simulink model "gm_minutiaeextraction_21821"  (R2018b)
settings: Solver=FixedStepDiscrete  StartTime=0.0  StopTime=10  RelTol=1e-3
undefined symbols (not defined in the file or in its folder): gray
libraries: hdlsllib x4, visionsources x1, dspmtrx3 x1
(part 5 of 7)

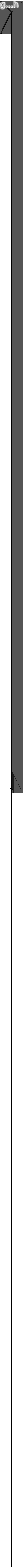
== system gm_minutiaeextraction_21821/MinutiaeFeature/MinutaeExtractTh ==
  In1 : Inport  OutDataTypeStr=boolean  PortDimensions=[128,64]  SampleTime=0.1
  MATLAB Function1 : Subsystem
  Serializer1D : hdlsllib/HDL Operations/Serializer1D  Ratio=8192  IdleCycles=0  validIn=off  startOut=off  validOut=off  inputDataDimensions=8192  inputSampleTime=0.1  inputSignalType=real
      settings: SourceProductName=HDL Coder  SourceProductBaseCode=HD
  concatenate : Concatenate  NumInputs=8192  ConcatenateDimension=2
  t : Subsystem
  t{1..64} (64 alike) : Demux  Outputs=128
  Out1 : Outport
  wires:
  In1/1 -> MATLAB Function1/1(X)
  MATLAB Function1/1(Y) -> t/1(in0)
  concatenate/1 -> Serializer1D/1
  Serializer1D/1 -> Out1/1
  t/1(out0) -> t1/1
  t/2(out1) -> t2/1
  t/3(out2) -> t3/1
  t/4(out3) -> t4/1
  t/5(out4) -> t5/1
  t/6(out5) -> t6/1
  t/7(out6) -> t7/1
  t/8(out7) -> t8/1
  t/9(out8) -> t9/1
  t/10(out9) -> t10/1
  t/11(out10) -> t11/1
  t/12(out11) -> t12/1
  t/13(out12) -> t13/1
  t/14(out13) -> t14/1
  t/15(out14) -> t15/1
  t/16(out15) -> t16/1
  t/17(out16) -> t17/1
  t/18(out17) -> t18/1
  t/19(out18) -> t19/1
  t/20(out19) -> t20/1
  t/21(out20) -> t21/1
  t/22(out21) -> t22/1
  t/23(out22) -> t23/1
  t/24(out23) -> t24/1
  t/25(out24) -> t25/1
  t/26(out25) -> t26/1
  t/27(out26) -> t27/1
  t/28(out27) -> t28/1
  t/29(out28) -> t29/1
  t/30(out29) -> t30/1
  t/31(out30) -> t31/1
  t/32(out31) -> t32/1
  t/33(out32) -> t33/1
  t/34(out33) -> t34/1
  t/35(out34) -> t35/1
  t/36(out35) -> t36/1
  t/37(out36) -> t37/1
  t/38(out37) -> t38/1
  t/39(out38) -> t39/1
  t/40(out39) -> t40/1
  t/41(out40) -> t41/1
  t/42(out41) -> t42/1
  t/43(out42) -> t43/1
  t/44(out43) -> t44/1
  t/45(out44) -> t45/1
  t/46(out45) -> t46/1
  t/47(out46) -> t47/1
  t/48(out47) -> t48/1
  t/49(out48) -> t49/1
  t/50(out49) -> t50/1
  t/51(out50) -> t51/1
  t/52(out51) -> t52/1
  t/53(out52) -> t53/1
  t/54(out53) -> t54/1
  t/55(out54) -> t55/1
  t/56(out55) -> t56/1
  t/57(out56) -> t57/1
  t/58(out57) -> t58/1
  t/59(out58) -> t59/1
  t/60(out59) -> t60/1
  t/61(out60) -> t61/1
  t/62(out61) -> t62/1
  t/63(out62) -> t63/1
  t/64(out63) -> t64/1
  t1/1 -> concatenate/1
  t1/2 -> concatenate/2
  t1/3 -> concatenate/3
  t1/4 -> concatenate/4
  t1/5 -> concatenate/5
  t1/6 -> concatenate/6
  t1/7 -> concatenate/7
  t1/8 -> concatenate/8
  t1/9 -> concatenate/9
  t1/10 -> concatenate/10
  t1/11 -> concatenate/11
  t1/12 -> concatenate/12
  t1/13 -> concatenate/13
  t1/14 -> concatenate/14
  t1/15 -> concatenate/15
  t1/16 -> concatenate/16
  t1/17 -> concatenate/17
  t1/18 -> concatenate/18
  t1/19 -> concatenate/19
  t1/20 -> concatenate/20
  t1/21 -> concatenate/21
  t1/22 -> concatenate/22
  t1/23 -> concatenate/23
  t1/24 -> concatenate/24
  t1/25 -> concatenate/25
  t1/26 -> concatenate/26
  t1/27 -> concatenate/27
  t1/28 -> concatenate/28
  t1/29 -> concatenate/29
  t1/30 -> concatenate/30
  t1/31 -> concatenate/31
  t1/32 -> concatenate/32
  t1/33 -> concatenate/33
  t1/34 -> concatenate/34
  t1/35 -> concatenate/35
  t1/36 -> concatenate/36
  t1/37 -> concatenate/37
  t1/38 -> concatenate/38
  t1/39 -> concatenate/39
  t1/40 -> concatenate/40
  t1/41 -> concatenate/41
  t1/42 -> concatenate/42
  t1/43 -> concatenate/43
  t1/44 -> concatenate/44
  t1/45 -> concatenate/45
  t1/46 -> concatenate/46
  t1/47 -> concatenate/47
  t1/48 -> concatenate/48
  t1/49 -> concatenate/49
  t1/50 -> concatenate/50
  t1/51 -> concatenate/51
  t1/52 -> concatenate/52
  t1/53 -> concatenate/53
  t1/54 -> concatenate/54
  t1/55 -> concatenate/55
  t1/56 -> concatenate/56
  t1/57 -> concatenate/57
  t1/58 -> concatenate/58
  t1/59 -> concatenate/59
  t1/60 -> concatenate/60
  t1/61 -> concatenate/61
  t1/62 -> concatenate/62
  t1/63 -> concatenate/63
  t1/64 -> concatenate/64
  t1/65 -> concatenate/65
  t1/66 -> concatenate/66
  t1/67 -> concatenate/67
  t1/68 -> concatenate/68
  t1/69 -> concatenate/69
  t1/70 -> concatenate/70
  t1/71 -> concatenate/71
  t1/72 -> concatenate/72
  t1/73 -> concatenate/73
  t1/74 -> concatenate/74
  t1/75 -> concatenate/75
  t1/76 -> concatenate/76
  t1/77 -> concatenate/77
  t1/78 -> concatenate/78
  t1/79 -> concatenate/79
  t1/80 -> concatenate/80
  t1/81 -> concatenate/81
  t1/82 -> concatenate/82
  t1/83 -> concatenate/83
  t1/84 -> concatenate/84
  t1/85 -> concatenate/85
  t1/86 -> concatenate/86
  t1/87 -> concatenate/87
  t1/88 -> concatenate/88
  t1/89 -> concatenate/89
  t1/90 -> concatenate/90
  t1/91 -> concatenate/91
  t1/92 -> concatenate/92
  t1/93 -> concatenate/93
  t1/94 -> concatenate/94
  t1/95 -> concatenate/95
  t1/96 -> concatenate/96
  t1/97 -> concatenate/97
  t1/98 -> concatenate/98
  t1/99 -> concatenate/99
  t1/100 -> concatenate/100
  t1/101 -> concatenate/101
  t1/102 -> concatenate/102
  t1/103 -> concatenate/103
  t1/104 -> concatenate/104
  t1/105 -> concatenate/105
  t1/106 -> concatenate/106
  t1/107 -> concatenate/107
  t1/108 -> concatenate/108
  t1/109 -> concatenate/109
  t1/110 -> concatenate/110
  t1/111 -> concatenate/111
  t1/112 -> concatenate/112
  t1/113 -> concatenate/113
  t1/114 -> concatenate/114
  t1/115 -> concatenate/115
  t1/116 -> concatenate/116
  t1/117 -> concatenate/117
  t1/118 -> concatenate/118
  t1/119 -> concatenate/119
  t1/120 -> concatenate/120
  t1/121 -> concatenate/121
  t1/122 -> concatenate/122
  t1/123 -> concatenate/123
  t1/124 -> concatenate/124
  t1/125 -> concatenate/125
  t1/126 -> concatenate/126
  t1/127 -> concatenate/127
  t1/128 -> concatenate/128
  t2/1 -> concatenate/129
  t2/2 -> concatenate/130
  t2/3 -> concatenate/131
  t2/4 -> concatenate/132
  t2/5 -> concatenate/133
  t2/6 -> concatenate/134
  t2/7 -> concatenate/135
  t2/8 -> concatenate/136
  t2/9 -> concatenate/137
  t2/10 -> concatenate/138
  t2/11 -> concatenate/139
  t2/12 -> concatenate/140
  t2/13 -> concatenate/141
  t2/14 -> concatenate/142
  t2/15 -> concatenate/143
  t2/16 -> concatenate/144
  t2/17 -> concatenate/145
  t2/18 -> concatenate/146
  t2/19 -> concatenate/147
  t2/20 -> concatenate/148
  t2/21 -> concatenate/149
  t2/22 -> concatenate/150
  t2/23 -> concatenate/151
  t2/24 -> concatenate/152
  t2/25 -> concatenate/153
  t2/26 -> concatenate/154
  t2/27 -> concatenate/155
  t2/28 -> concatenate/156
  t2/29 -> concatenate/157
  t2/30 -> concatenate/158
  t2/31 -> concatenate/159
  t2/32 -> concatenate/160
  t2/33 -> concatenate/161
  t2/34 -> concatenate/162
  t2/35 -> concatenate/163
  t2/36 -> concatenate/164
  t2/37 -> concatenate/165
  t2/38 -> concatenate/166
  t2/39 -> concatenate/167
  t2/40 -> concatenate/168
  t2/41 -> concatenate/169
  t2/42 -> concatenate/170
  t2/43 -> concatenate/171
  t2/44 -> concatenate/172
  t2/45 -> concatenate/173
  t2/46 -> concatenate/174
  t2/47 -> concatenate/175
  t2/48 -> concatenate/176
  t2/49 -> concatenate/177
  t2/50 -> concatenate/178
  t2/51 -> concatenate/179
  t2/52 -> concatenate/180
  t2/53 -> concatenate/181
  t2/54 -> concatenate/182
  t2/55 -> concatenate/183
  t2/56 -> concatenate/184
  t2/57 -> concatenate/185
  t2/58 -> concatenate/186
  t2/59 -> concatenate/187
  t2/60 -> concatenate/188
  t2/61 -> concatenate/189
  t2/62 -> concatenate/190
  t2/63 -> concatenate/191
  t2/64 -> concatenate/192
  t2/65 -> concatenate/193
  t2/66 -> concatenate/194
  t2/67 -> concatenate/195
  t2/68 -> concatenate/196
  t2/69 -> concatenate/197
  t2/70 -> concatenate/198
  t2/71 -> concatenate/199
  t2/72 -> concatenate/200
  t2/73 -> concatenate/201
  t2/74 -> concatenate/202
  t2/75 -> concatenate/203
  t2/76 -> concatenate/204
  t2/77 -> concatenate/205
  t2/78 -> concatenate/206
  t2/79 -> concatenate/207
  t2/80 -> concatenate/208
  t2/81 -> concatenate/209
  t2/82 -> concatenate/210
  t2/83 -> concatenate/211
  t2/84 -> concatenate/212
  t2/85 -> concatenate/213
  t2/86 -> concatenate/214
  t2/87 -> concatenate/215
  t2/88 -> concatenate/216
  t2/89 -> concatenate/217
  t2/90 -> concatenate/218
  t2/91 -> concatenate/219
  t2/92 -> concatenate/220
  t2/93 -> concatenate/221
  t2/94 -> concatenate/222
  t2/95 -> concatenate/223
  t2/96 -> concatenate/224
  t2/97 -> concatenate/225
  t2/98 -> concatenate/226
  t2/99 -> concatenate/227
  t2/100 -> concatenate/228
  t2/101 -> concatenate/229
  t2/102 -> concatenate/230
  t2/103 -> concatenate/231
  t2/104 -> concatenate/232
  t2/105 -> concatenate/233
  t2/106 -> concatenate/234
  t2/107 -> concatenate/235
  t2/108 -> concatenate/236
  t2/109 -> concatenate/237
  t2/110 -> concatenate/238
  t2/111 -> concatenate/239
  t2/112 -> concatenate/240
  t2/113 -> concatenate/241
  t2/114 -> concatenate/242
  t2/115 -> concatenate/243
  t2/116 -> concatenate/244
  t2/117 -> concatenate/245
  t2/118 -> concatenate/246
  t2/119 -> concatenate/247
  t2/120 -> concatenate/248
  t2/121 -> concatenate/249
  t2/122 -> concatenate/250
  t2/123 -> concatenate/251
  t2/124 -> concatenate/252
  t2/125 -> concatenate/253
  t2/126 -> concatenate/254
  t2/127 -> concatenate/255
  t2/128 -> concatenate/256
  t3/1 -> concatenate/257
  t3/2 -> concatenate/258
  t3/3 -> concatenate/259
  t3/4 -> concatenate/260
  t3/5 -> concatenate/261
  t3/6 -> concatenate/262
  t3/7 -> concatenate/263
  t3/8 -> concatenate/264
  t3/9 -> concatenate/265
  t3/10 -> concatenate/266
  t3/11 -> concatenate/267
  t3/12 -> concatenate/268
  t3/13 -> concatenate/269
  t3/14 -> concatenate/270
  t3/15 -> concatenate/271
  t3/16 -> concatenate/272
  t3/17 -> concatenate/273
  t3/18 -> concatenate/274
  t3/19 -> concatenate/275
  t3/20 -> concatenate/276
  t3/21 -> concatenate/277
  t3/22 -> concatenate/278
  t3/23 -> concatenate/279
  t3/24 -> concatenate/280
  t3/25 -> concatenate/281
  t3/26 -> concatenate/282
  t3/27 -> concatenate/283
  t3/28 -> concatenate/284
  t3/29 -> concatenate/285
  t3/30 -> concatenate/286
  t3/31 -> concatenate/287
  t3/32 -> concatenate/288
  t3/33 -> concatenate/289
  t3/34 -> concatenate/290
  t3/35 -> concatenate/291
  t3/36 -> concatenate/292
  t3/37 -> concatenate/293
  t3/38 -> concatenate/294
  t3/39 -> concatenate/295
  t3/40 -> concatenate/296
  t3/41 -> concatenate/297
  t3/42 -> concatenate/298
  t3/43 -> concatenate/299
  t3/44 -> concatenate/300
  t3/45 -> concatenate/301
  t3/46 -> concatenate/302
  t3/47 -> concatenate/303
  t3/48 -> concatenate/304
  t3/49 -> concatenate/305
  t3/50 -> concatenate/306
  t3/51 -> concatenate/307
  t3/52 -> concatenate/308
  t3/53 -> concatenate/309
  t3/54 -> concatenate/310
  t3/55 -> concatenate/311
  t3/56 -> concatenate/312
  t3/57 -> concatenate/313
  t3/58 -> concatenate/314
  t3/59 -> concatenate/315
  t3/60 -> concatenate/316
  t3/61 -> concatenate/317
  t3/62 -> concatenate/318
  t3/63 -> concatenate/319
  t3/64 -> concatenate/320
  t3/65 -> concatenate/321
  t3/66 -> concatenate/322
  t3/67 -> concatenate/323
  t3/68 -> concatenate/324
  t3/69 -> concatenate/325
  t3/70 -> concatenate/326
  t3/71 -> concatenate/327
  t3/72 -> concatenate/328
  t3/73 -> concatenate/329
  t3/74 -> concatenate/330
  t3/75 -> concatenate/331
  t3/76 -> concatenate/332
  t3/77 -> concatenate/333
  t3/78 -> concatenate/334
  t3/79 -> concatenate/335
  t3/80 -> concatenate/336
  t3/81 -> concatenate/337
  t3/82 -> concatenate/338
  t3/83 -> concatenate/339
  t3/84 -> concatenate/340
  t3/85 -> concatenate/341
  t3/86 -> concatenate/342
  t3/87 -> concatenate/343
  t3/88 -> concatenate/344
  t3/89 -> concatenate/345
  t3/90 -> concatenate/346
  t3/91 -> concatenate/347
  t3/92 -> concatenate/348
  t3/93 -> concatenate/349
  t3/94 -> concatenate/350
  t3/95 -> concatenate/351
  t3/96 -> concatenate/352
  t3/97 -> concatenate/353
  t3/98 -> concatenate/354
  t3/99 -> concatenate/355
  t3/100 -> concatenate/356
  t3/101 -> concatenate/357
  t3/102 -> concatenate/358
  t3/103 -> concatenate/359
  t3/104 -> concatenate/360
  t3/105 -> concatenate/361
  t3/106 -> concatenate/362
  t3/107 -> concatenate/363
  t3/108 -> concatenate/364
  t3/109 -> concatenate/365
  t3/110 -> concatenate/366
  t3/111 -> concatenate/367
  t3/112 -> concatenate/368
  t3/113 -> concatenate/369
  t3/114 -> concatenate/370
  t3/115 -> concatenate/371
  t3/116 -> concatenate/372
  t3/117 -> concatenate/373
  t3/118 -> concatenate/374
  t3/119 -> concatenate/375
  t3/120 -> concatenate/376
  t3/121 -> concatenate/377
  t3/122 -> concatenate/378
  t3/123 -> concatenate/379
  t3/124 -> concatenate/380
  t3/125 -> concatenate/381
  t3/126 -> concatenate/382
  t3/127 -> concatenate/383
  t3/128 -> concatenate/384
  t4/1 -> concatenate/385
  t4/2 -> concatenate/386
  t4/3 -> concatenate/387
  t4/4 -> concatenate/388
  t4/5 -> concatenate/389
  t4/6 -> concatenate/390
  t4/7 -> concatenate/391
  t4/8 -> concatenate/392
  t4/9 -> concatenate/393
  t4/10 -> concatenate/394
  t4/11 -> concatenate/395
  t4/12 -> concatenate/396
  t4/13 -> concatenate/397
  t4/14 -> concatenate/398
  t4/15 -> concatenate/399
  t4/16 -> concatenate/400
  t4/17 -> concatenate/401
  t4/18 -> concatenate/402
  t4/19 -> concatenate/403
  t4/20 -> concatenate/404
  t4/21 -> concatenate/405
  t4/22 -> concatenate/406
  t4/23 -> concatenate/407
  t4/24 -> concatenate/408
  t4/25 -> concatenate/409
  t4/26 -> concatenate/410
  t4/27 -> concatenate/411
  t4/28 -> concatenate/412
  t4/29 -> concatenate/413
  t4/30 -> concatenate/414
  t4/31 -> concatenate/415
  t4/32 -> concatenate/416
  t4/33 -> concatenate/417
  t4/34 -> concatenate/418
  t4/35 -> concatenate/419
  t4/36 -> concatenate/420
  t4/37 -> concatenate/421
  t4/38 -> concatenate/422
  t4/39 -> concatenate/423
  t4/40 -> concatenate/424
  t4/41 -> concatenate/425
  t4/42 -> concatenate/426
  t4/43 -> concatenate/427
  t4/44 -> concatenate/428
  t4/45 -> concatenate/429
  t4/46 -> concatenate/430
  t4/47 -> concatenate/431
  t4/48 -> concatenate/432
  t4/49 -> concatenate/433
  t4/50 -> concatenate/434
  t4/51 -> concatenate/435
  t4/52 -> concatenate/436
  t4/53 -> concatenate/437
  t4/54 -> concatenate/438
  t4/55 -> concatenate/439
  t4/56 -> concatenate/440
  t4/57 -> concatenate/441
  t4/58 -> concatenate/442
  t4/59 -> concatenate/443
  t4/60 -> concatenate/444
  t4/61 -> concatenate/445
  t4/62 -> concatenate/446
  t4/63 -> concatenate/447
  t4/64 -> concatenate/448
  t4/65 -> concatenate/449
  t4/66 -> concatenate/450
  t4/67 -> concatenate/451
  t4/68 -> concatenate/452
  t4/69 -> concatenate/453
  t4/70 -> concatenate/454
  t4/71 -> concatenate/455
  t4/72 -> concatenate/456
  t4/73 -> concatenate/457
  t4/74 -> concatenate/458
  t4/75 -> concatenate/459
  t4/76 -> concatenate/460
  t4/77 -> concatenate/461
  t4/78 -> concatenate/462
  t4/79 -> concatenate/463
  t4/80 -> concatenate/464
  t4/81 -> concatenate/465
  t4/82 -> concatenate/466
  t4/83 -> concatenate/467
  t4/84 -> concatenate/468
  t4/85 -> concatenate/469
  t4/86 -> concatenate/470
  t4/87 -> concatenate/471
  t4/88 -> concatenate/472
  t4/89 -> concatenate/473
  t4/90 -> concatenate/474
  t4/91 -> concatenate/475
  t4/92 -> concatenate/476
  t4/93 -> concatenate/477
  t4/94 -> concatenate/478
  t4/95 -> concatenate/479
  t4/96 -> concatenate/480
  t4/97 -> concatenate/481
  t4/98 -> concatenate/482
  t4/99 -> concatenate/483
  t4/100 -> concatenate/484
  t4/101 -> concatenate/485
  t4/102 -> concatenate/486
  t4/103 -> concatenate/487
  t4/104 -> concatenate/488
  t4/105 -> concatenate/489
  t4/106 -> concatenate/490
  t4/107 -> concatenate/491
  t4/108 -> concatenate/492
  t4/109 -> concatenate/493
  t4/110 -> concatenate/494
  t4/111 -> concatenate/495
  t4/112 -> concatenate/496
  t4/113 -> concatenate/497
  t4/114 -> concatenate/498
  t4/115 -> concatenate/499
  t4/116 -> concatenate/500
  t4/117 -> concatenate/501
  t4/118 -> concatenate/502
  t4/119 -> concatenate/503
  t4/120 -> concatenate/504
  t4/121 -> concatenate/505
  t4/122 -> concatenate/506
  t4/123 -> concatenate/507
  t4/124 -> concatenate/508
  t4/125 -> concatenate/509
  t4/126 -> concatenate/510
  t4/127 -> concatenate/511
  t4/128 -> concatenate/512
  t5/1 -> concatenate/513
  t5/2 -> concatenate/514
  t5/3 -> concatenate/515
  t5/4 -> concatenate/516
  t5/5 -> concatenate/517
  t5/6 -> concatenate/518
  t5/7 -> concatenate/519
  t5/8 -> concatenate/520
  t5/9 -> concatenate/521
  t5/10 -> concatenate/522
  t5/11 -> concatenate/523
  t5/12 -> concatenate/524
  t5/13 -> concatenate/525
  t5/14 -> concatenate/526
  t5/15 -> concatenate/527
  t5/16 -> concatenate/528
  t5/17 -> concatenate/529
  t5/18 -> concatenate/530
  t5/19 -> concatenate/531
  t5/20 -> concatenate/532
  t5/21 -> concatenate/533
  t5/22 -> concatenate/534
  t5/23 -> concatenate/535
  t5/24 -> concatenate/536
  t5/25 -> concatenate/537
  t5/26 -> concatenate/538
  t5/27 -> concatenate/539
  t5/28 -> concatenate/540
  t5/29 -> concatenate/541
  t5/30 -> concatenate/542
  t5/31 -> concatenate/543
  t5/32 -> concatenate/544
  t5/33 -> concatenate/545
  t5/34 -> concatenate/546
  t5/35 -> concatenate/547
  t5/36 -> concatenate/548
  t5/37 -> concatenate/549
  t5/38 -> concatenate/550
  t5/39 -> concatenate/551
  t5/40 -> concatenate/552
  t5/41 -> concatenate/553
  t5/42 -> concatenate/554
  t5/43 -> concatenate/555
  t5/44 -> concatenate/556
  t5/45 -> concatenate/557
  t5/46 -> concatenate/558
  t5/47 -> concatenate/559
  t5/48 -> concatenate/560
  t5/49 -> concatenate/561
  t5/50 -> concatenate/562
  t5/51 -> concatenate/563
  t5/52 -> concatenate/564
  t5/53 -> concatenate/565
  t5/54 -> concatenate/566
  t5/55 -> concatenate/567
  t5/56 -> concatenate/568
  t5/57 -> concatenate/569
  t5/58 -> concatenate/570
  t5/59 -> concatenate/571
  t5/60 -> concatenate/572
  t5/61 -> concatenate/573
  t5/62 -> concatenate/574
  t5/63 -> concatenate/575
  t5/64 -> concatenate/576
  t5/65 -> concatenate/577
  t5/66 -> concatenate/578
  t5/67 -> concatenate/579
  t5/68 -> concatenate/580
  t5/69 -> concatenate/581
  t5/70 -> concatenate/582
  t5/71 -> concatenate/583
  t5/72 -> concatenate/584
  t5/73 -> concatenate/585
  t5/74 -> concatenate/586
  t5/75 -> concatenate/587
  t5/76 -> concatenate/588
  t5/77 -> concatenate/589
  t5/78 -> concatenate/590
  t5/79 -> concatenate/591
  t5/80 -> concatenate/592
  t5/81 -> concatenate/593
  t5/82 -> concatenate/594
  t5/83 -> concatenate/595
  t5/84 -> concatenate/596
  t5/85 -> concatenate/597
  t5/86 -> concatenate/598
  t5/87 -> concatenate/599
  t5/88 -> concatenate/600
  t5/89 -> concatenate/601
  t5/90 -> concatenate/602
  t5/91 -> concatenate/603
  t5/92 -> concatenate/604
  t5/93 -> concatenate/605
  t5/94 -> concatenate/606
  t5/95 -> concatenate/607
  t5/96 -> concatenate/608
  t5/97 -> concatenate/609
  t5/98 -> concatenate/610
  t5/99 -> concatenate/611
  t5/100 -> concatenate/612
  t5/101 -> concatenate/613
  t5/102 -> concatenate/614
  t5/103 -> concatenate/615
  t5/104 -> concatenate/616
  t5/105 -> concatenate/617
  t5/106 -> concatenate/618
  t5/107 -> concatenate/619
  t5/108 -> concatenate/620
  t5/109 -> concatenate/621
  t5/110 -> concatenate/622
  t5/111 -> concatenate/623
  t5/112 -> concatenate/624
  t5/113 -> concatenate/625
  t5/114 -> concatenate/626
  t5/115 -> concatenate/627
  t5/116 -> concatenate/628
  t5/117 -> concatenate/629
  t5/118 -> concatenate/630
  t5/119 -> concatenate/631
  t5/120 -> concatenate/632
  t5/121 -> concatenate/633
  t5/122 -> concatenate/634
  t5/123 -> concatenate/635
  t5/124 -> concatenate/636
  t5/125 -> concatenate/637
  t5/126 -> concatenate/638
  t5/127 -> concatenate/639
  t5/128 -> concatenate/640
  t6/1 -> concatenate/641
  t6/2 -> concatenate/642
  t6/3 -> concatenate/643
  t6/4 -> concatenate/644
  t6/5 -> concatenate/645
  t6/6 -> concatenate/646
  t6/7 -> concatenate/647
  t6/8 -> concatenate/648
  t6/9 -> concatenate/649
  t6/10 -> concatenate/650
  t6/11 -> concatenate/651
  t6/12 -> concatenate/652
  t6/13 -> concatenate/653
  t6/14 -> concatenate/654
  t6/15 -> concatenate/655
  t6/16 -> concatenate/656
  t6/17 -> concatenate/657
  t6/18 -> concatenate/658
  t6/19 -> concatenate/659
  t6/20 -> concatenate/660
  t6/21 -> concatenate/661
  t6/22 -> concatenate/662
  t6/23 -> concatenate/663
  t6/24 -> concatenate/664
  t6/25 -> concatenate/665
  t6/26 -> concatenate/666
  t6/27 -> concatenate/667
  t6/28 -> concatenate/668
  t6/29 -> concatenate/669
  t6/30 -> concatenate/670
  t6/31 -> concatenate/671
  t6/32 -> concatenate/672
  t6/33 -> concatenate/673
  t6/34 -> concatenate/674
  t6/35 -> concatenate/675
  t6/36 -> concatenate/676
  t6/37 -> concatenate/677
  t6/38 -> concatenate/678
  t6/39 -> concatenate/679
  t6/40 -> concatenate/680
  t6/41 -> concatenate/681
  t6/42 -> concatenate/682
  t6/43 -> concatenate/683
  t6/44 -> concatenate/684
  t6/45 -> concatenate/685
  t6/46 -> concatenate/686
  t6/47 -> concatenate/687
  t6/48 -> concatenate/688
  t6/49 -> concatenate/689
  t6/50 -> concatenate/690
  t6/51 -> concatenate/691
  t6/52 -> concatenate/692
  t6/53 -> concatenate/693
  t6/54 -> concatenate/694
  t6/55 -> concatenate/695
  t6/56 -> concatenate/696
  t6/57 -> concatenate/697
  t6/58 -> concatenate/698
  t6/59 -> concatenate/699
  t6/60 -> concatenate/700
  t6/61 -> concatenate/701
  t6/62 -> concatenate/702
  t6/63 -> concatenate/703
  t6/64 -> concatenate/704
  t6/65 -> concatenate/705
  t6/66 -> concatenate/706
  t6/67 -> concatenate/707
  t6/68 -> concatenate/708
  t6/69 -> concatenate/709
  t6/70 -> concatenate/710
  t6/71 -> concatenate/711
  t6/72 -> concatenate/712
  t6/73 -> concatenate/713
  t6/74 -> concatenate/714
  t6/75 -> concatenate/715
  t6/76 -> concatenate/716
  t6/77 -> concatenate/717
  t6/78 -> concatenate/718
  t6/79 -> concatenate/719
  t6/80 -> concatenate/720
  t6/81 -> concatenate/721
  t6/82 -> concatenate/722
  t6/83 -> concatenate/723
  t6/84 -> concatenate/724
  t6/85 -> concatenate/725
  t6/86 -> concatenate/726
  t6/87 -> concatenate/727
  t6/88 -> concatenate/728
  t6/89 -> concatenate/729
  t6/90 -> concatenate/730
  t6/91 -> concatenate/731
  t6/92 -> concatenate/732
  t6/93 -> concatenate/733
  t6/94 -> concatenate/734
  t6/95 -> concatenate/735
  t6/96 -> concatenate/736
  t6/97 -> concatenate/737
  t6/98 -> concatenate/738
  t6/99 -> concatenate/739
  t6/100 -> concatenate/740
  t6/101 -> concatenate/741
  t6/102 -> concatenate/742
  t6/103 -> concatenate/743
  t6/104 -> concatenate/744
  t6/105 -> concatenate/745
  t6/106 -> concatenate/746
  t6/107 -> concatenate/747
  t6/108 -> concatenate/748
  t6/109 -> concatenate/749
  t6/110 -> concatenate/750
  t6/111 -> concatenate/751
  t6/112 -> concatenate/752
  t6/113 -> concatenate/753
  t6/114 -> concatenate/754
  t6/115 -> concatenate/755
  t6/116 -> concatenate/756
  t6/117 -> concatenate/757
  t6/118 -> concatenate/758
  t6/119 -> concatenate/759
  t6/120 -> concatenate/760
  t6/121 -> concatenate/761
  t6/122 -> concatenate/762
  t6/123 -> concatenate/763
  t6/124 -> concatenate/764
  t6/125 -> concatenate/765
  t6/126 -> concatenate/766
  t6/127 -> concatenate/767
  t6/128 -> concatenate/768
  t7/1 -> concatenate/769
  t7/2 -> concatenate/770
  t7/3 -> concatenate/771
  t7/4 -> concatenate/772
  t7/5 -> concatenate/773
  t7/6 -> concatenate/774
  t7/7 -> concatenate/775
  t7/8 -> concatenate/776
  t7/9 -> concatenate/777
  t7/10 -> concatenate/778
  t7/11 -> concatenate/779
  t7/12 -> concatenate/780
  t7/13 -> concatenate/781
  t7/14 -> concatenate/782
  t7/15 -> concatenate/783
  t7/16 -> concatenate/784
  t7/17 -> concatenate/785
  t7/18 -> concatenate/786
  t7/19 -> concatenate/787
  t7/20 -> concatenate/788
  t7/21 -> concatenate/789
  t7/22 -> concatenate/790
  t7/23 -> concatenate/791
  t7/24 -> concatenate/792
  t7/25 -> concatenate/793
  t7/26 -> concatenate/794
  t7/27 -> concatenate/795
  t7/28 -> concatenate/796
  t7/29 -> concatenate/797
  t7/30 -> concatenate/798
  t7/31 -> concatenate/799
  t7/32 -> concatenate/800
  t7/33 -> concatenate/801
  t7/34 -> concatenate/802
  t7/35 -> concatenate/803
  t7/36 -> concatenate/804
  t7/37 -> concatenate/805
  t7/38 -> concatenate/806
  t7/39 -> concatenate/807
  t7/40 -> concatenate/808
  t7/41 -> concatenate/809
  t7/42 -> concatenate/810
  t7/43 -> concatenate/811
  t7/44 -> concatenate/812
  t7/45 -> concatenate/813
  t7/46 -> concatenate/814
  t7/47 -> concatenate/815
  t7/48 -> concatenate/816
  t7/49 -> concatenate/817
  t7/50 -> concatenate/818
  t7/51 -> concatenate/819
  t7/52 -> concatenate/820
  t7/53 -> concatenate/821
  t7/54 -> concatenate/822
  t7/55 -> concatenate/823
  t7/56 -> concatenate/824
  t7/57 -> concatenate/825
  t7/58 -> concatenate/826
  t7/59 -> concatenate/827
  t7/60 -> concatenate/828
  t7/61 -> concatenate/829
  t7/62 -> concatenate/830
  t7/63 -> concatenate/831
  t7/64 -> concatenate/832
  t7/65 -> concatenate/833
  t7/66 -> concatenate/834
  t7/67 -> concatenate/835
  t7/68 -> concatenate/836
  t7/69 -> concatenate/837
  t7/70 -> concatenate/838
  t7/71 -> concatenate/839
  t7/72 -> concatenate/840
  t7/73 -> concatenate/841
  t7/74 -> concatenate/842
  t7/75 -> concatenate/843
  t7/76 -> concatenate/844
  t7/77 -> concatenate/845
  t7/78 -> concatenate/846
  t7/79 -> concatenate/847
  t7/80 -> concatenate/848
  t7/81 -> concatenate/849
  t7/82 -> concatenate/850
  t7/83 -> concatenate/851
  t7/84 -> concatenate/852
  t7/85 -> concatenate/853
  t7/86 -> concatenate/854
  t7/87 -> concatenate/855
  t7/88 -> concatenate/856
  t7/89 -> concatenate/857
  t7/90 -> concatenate/858
  t7/91 -> concatenate/859
  t7/92 -> concatenate/860
  t7/93 -> concatenate/861
  t7/94 -> concatenate/862
  t7/95 -> concatenate/863
  t7/96 -> concatenate/864
  t7/97 -> concatenate/865
  t7/98 -> concatenate/866
  t7/99 -> concatenate/867
  t7/100 -> concatenate/868
  t7/101 -> concatenate/869
  t7/102 -> concatenate/870
  t7/103 -> concatenate/871
  t7/104 -> concatenate/872
  t7/105 -> concatenate/873
  t7/106 -> concatenate/874
  t7/107 -> concatenate/875
  t7/108 -> concatenate/876
  t7/109 -> concatenate/877
  t7/110 -> concatenate/878
  t7/111 -> concatenate/879
  t7/112 -> concatenate/880
  t7/113 -> concatenate/881
  t7/114 -> concatenate/882
  t7/115 -> concatenate/883
  t7/116 -> concatenate/884
  t7/117 -> concatenate/885
  t7/118 -> concatenate/886
  t7/119 -> concatenate/887
  t7/120 -> concatenate/888
  t7/121 -> concatenate/889
  t7/122 -> concatenate/890
  t7/123 -> concatenate/891
  t7/124 -> concatenate/892
  t7/125 -> concatenate/893
  t7/126 -> concatenate/894
  t7/127 -> concatenate/895
  t7/128 -> concatenate/896
  t8/1 -> concatenate/897
  t8/2 -> concatenate/898
  t8/3 -> concatenate/899
  t8/4 -> concatenate/900
  t8/5 -> concatenate/901
  t8/6 -> concatenate/902
  t8/7 -> concatenate/903
  t8/8 -> concatenate/904
  t8/9 -> concatenate/905
  t8/10 -> concatenate/906
  t8/11 -> concatenate/907
  t8/12 -> concatenate/908
  t8/13 -> concatenate/909
  t8/14 -> concatenate/910
  t8/15 -> concatenate/911
  t8/16 -> concatenate/912
  t8/17 -> concatenate/913
  t8/18 -> concatenate/914
  t8/19 -> concatenate/915
  t8/20 -> concatenate/916
  t8/21 -> concatenate/917
  t8/22 -> concatenate/918
  t8/23 -> concatenate/919
  t8/24 -> concatenate/920
  t8/25 -> concatenate/921
  t8/26 -> concatenate/922
  t8/27 -> concatenate/923
  t8/28 -> concatenate/924
  t8/29 -> concatenate/925
  t8/30 -> concatenate/926
  t8/31 -> concatenate/927
  t8/32 -> concatenate/928
  t8/33 -> concatenate/929
  t8/34 -> concatenate/930
  t8/35 -> concatenate/931
  t8/36 -> concatenate/932
  t8/37 -> concatenate/933
  t8/38 -> concatenate/934
  t8/39 -> concatenate/935
  t8/40 -> concatenate/936
  t8/41 -> concatenate/937
  t8/42 -> concatenate/938
  t8/43 -> concatenate/939
  t8/44 -> concatenate/940
  t8/45 -> concatenate/941
  t8/46 -> concatenate/942
  t8/47 -> concatenate/943
  t8/48 -> concatenate/944
  t8/49 -> concatenate/945
  t8/50 -> concatenate/946
  t8/51 -> concatenate/947
  t8/52 -> concatenate/948
  t8/53 -> concatenate/949
  t8/54 -> concatenate/950
  t8/55 -> concatenate/951
  t8/56 -> concatenate/952
  t8/57 -> concatenate/953
  t8/58 -> concatenate/954
  t8/59 -> concatenate/955
  t8/60 -> concatenate/956
  t8/61 -> concatenate/957
  t8/62 -> concatenate/958
  t8/63 -> concatenate/959
  t8/64 -> concatenate/960
  t8/65 -> concatenate/961
  t8/66 -> concatenate/962
  t8/67 -> concatenate/963
  t8/68 -> concatenate/964
  t8/69 -> concatenate/965
  t8/70 -> concatenate/966
  t8/71 -> concatenate/967
  t8/72 -> concatenate/968
  t8/73 -> concatenate/969
  t8/74 -> concatenate/970
  t8/75 -> concatenate/971
  t8/76 -> concatenate/972
  t8/77 -> concatenate/973
  t8/78 -> concatenate/974
  t8/79 -> concatenate/975
  t8/80 -> concatenate/976
  t8/81 -> concatenate/977
  t8/82 -> concatenate/978
  t8/83 -> concatenate/979
  t8/84 -> concatenate/980
  t8/85 -> concatenate/981
  t8/86 -> concatenate/982
  t8/87 -> concatenate/983
  t8/88 -> concatenate/984
  t8/89 -> concatenate/985
  t8/90 -> concatenate/986
  t8/91 -> concatenate/987
  t8/92 -> concatenate/988
  t8/93 -> concatenate/989
  t8/94 -> concatenate/990
  t8/95 -> concatenate/991
  t8/96 -> concatenate/992
  t8/97 -> concatenate/993
  t8/98 -> concatenate/994
  t8/99 -> concatenate/995
  t8/100 -> concatenate/996
  t8/101 -> concatenate/997
  t8/102 -> concatenate/998
  t8/103 -> concatenate/999
  t8/104 -> concatenate/1000
  t8/105 -> concatenate/1001
  t8/106 -> concatenate/1002
  t8/107 -> concatenate/1003
  t8/108 -> concatenate/1004
  t8/109 -> concatenate/1005
  t8/110 -> concatenate/1006
  t8/111 -> concatenate/1007
  t8/112 -> concatenate/1008
  t8/113 -> concatenate/1009
  t8/114 -> concatenate/1010
  t8/115 -> concatenate/1011
  t8/116 -> concatenate/1012
  t8/117 -> concatenate/1013
  t8/118 -> concatenate/1014
  t8/119 -> concatenate/1015
  t8/120 -> concatenate/1016
  t8/121 -> concatenate/1017
  t8/122 -> concatenate/1018
  t8/123 -> concatenate/1019
  t8/124 -> concatenate/1020
  t8/125 -> concatenate/1021
  t8/126 -> concatenate/1022
  t8/127 -> concatenate/1023
  t8/128 -> concatenate/1024
  t9/1 -> concatenate/1025
  t9/2 -> concatenate/1026
  t9/3 -> concatenate/1027
  t9/4 -> concatenate/1028
  t9/5 -> concatenate/1029
  t9/6 -> concatenate/1030
  t9/7 -> concatenate/1031
  t9/8 -> concatenate/1032
  t9/9 -> concatenate/1033
  t9/10 -> concatenate/1034
  t9/11 -> concatenate/1035
  t9/12 -> concatenate/1036
  t9/13 -> concatenate/1037
  t9/14 -> concatenate/1038
  t9/15 -> concatenate/1039
  t9/16 -> concatenate/1040
  t9/17 -> concatenate/1041
  t9/18 -> concatenate/1042
  t9/19 -> concatenate/1043
  t9/20 -> concatenate/1044
  t9/21 -> concatenate/1045
  t9/22 -> concatenate/1046
  t9/23 -> concatenate/1047
  t9/24 -> concatenate/1048
  t9/25 -> concatenate/1049
  t9/26 -> concatenate/1050
  t9/27 -> concatenate/1051
  t9/28 -> concatenate/1052
  t9/29 -> concatenate/1053
  t9/30 -> concatenate/1054
  t9/31 -> concatenate/1055
  t9/32 -> concatenate/1056
  t9/33 -> concatenate/1057
  t9/34 -> concatenate/1058
  t9/35 -> concatenate/1059
  t9/36 -> concatenate/1060
  t9/37 -> concatenate/1061
  t9/38 -> concatenate/1062
  t9/39 -> concatenate/1063
  t9/40 -> concatenate/1064
  t9/41 -> concatenate/1065
  t9/42 -> concatenate/1066
  t9/43 -> concatenate/1067
  t9/44 -> concatenate/1068
  t9/45 -> concatenate/1069
  t9/46 -> concatenate/1070
  t9/47 -> concatenate/1071
  t9/48 -> concatenate/1072
  t9/49 -> concatenate/1073
  t9/50 -> concatenate/1074
  t9/51 -> concatenate/1075
  t9/52 -> concatenate/1076
  t9/53 -> concatenate/1077
  t9/54 -> concatenate/1078
  t9/55 -> concatenate/1079
  t9/56 -> concatenate/1080
  t9/57 -> concatenate/1081
  t9/58 -> concatenate/1082
  t9/59 -> concatenate/1083
  t9/60 -> concatenate/1084
  t9/61 -> concatenate/1085
  t9/62 -> concatenate/1086
  t9/63 -> concatenate/1087
  t9/64 -> concatenate/1088
  t9/65 -> concatenate/1089
  t9/66 -> concatenate/1090
  t9/67 -> concatenate/1091
  t9/68 -> concatenate/1092
  t9/69 -> concatenate/1093
  t9/70 -> concatenate/1094
  t9/71 -> concatenate/1095
  t9/72 -> concatenate/1096
  t9/73 -> concatenate/1097
  t9/74 -> concatenate/1098
  t9/75 -> concatenate/1099
  t9/76 -> concatenate/1100
  t9/77 -> concatenate/1101
  t9/78 -> concatenate/1102
  t9/79 -> concatenate/1103
  t9/80 -> concatenate/1104
  t9/81 -> concatenate/1105
  t9/82 -> concatenate/1106
  t9/83 -> concatenate/1107
  t9/84 -> concatenate/1108
  t9/85 -> concatenate/1109
  t9/86 -> concatenate/1110
  t9/87 -> concatenate/1111
  t9/88 -> concatenate/1112
  t9/89 -> concatenate/1113
  t9/90 -> concatenate/1114
  t9/91 -> concatenate/1115
  t9/92 -> concatenate/1116
  t9/93 -> concatenate/1117
  t9/94 -> concatenate/1118
  t9/95 -> concatenate/1119
  t9/96 -> concatenate/1120
  t9/97 -> concatenate/1121
  t9/98 -> concatenate/1122
  t9/99 -> concatenate/1123
  t9/100 -> concatenate/1124
  t9/101 -> concatenate/1125
  t9/102 -> concatenate/1126
  t9/103 -> concatenate/1127
  t9/104 -> concatenate/1128
  t9/105 -> concatenate/1129
  t9/106 -> concatenate/1130
  t9/107 -> concatenate/1131
  t9/108 -> concatenate/1132
  t9/109 -> concatenate/1133
  t9/110 -> concatenate/1134
  t9/111 -> concatenate/1135
  t9/112 -> concatenate/1136
  t9/113 -> concatenate/1137
  t9/114 -> concatenate/1138
  t9/115 -> concatenate/1139
  t9/116 -> concatenate/1140
  t9/117 -> concatenate/1141
  t9/118 -> concatenate/1142
  t9/119 -> concatenate/1143
  t9/120 -> concatenate/1144
  t9/121 -> concatenate/1145
  t9/122 -> concatenate/1146
  t9/123 -> concatenate/1147
  t9/124 -> concatenate/1148
  t9/125 -> concatenate/1149
  t9/126 -> concatenate/1150
  t9/127 -> concatenate/1151
  t9/128 -> concatenate/1152
  t10/1 -> concatenate/1153
  t10/2 -> concatenate/1154
  t10/3 -> concatenate/1155
  t10/4 -> concatenate/1156
  t10/5 -> concatenate/1157
  t10/6 -> concatenate/1158
  t10/7 -> concatenate/1159
  t10/8 -> concatenate/1160
  t10/9 -> concatenate/1161
  t10/10 -> concatenate/1162
  t10/11 -> concatenate/1163
  t10/12 -> concatenate/1164
  t10/13 -> concatenate/1165
  t10/14 -> concatenate/1166
  t10/15 -> concatenate/1167
  t10/16 -> concatenate/1168
  t10/17 -> concatenate/1169
  t10/18 -> concatenate/1170
  t10/19 -> concatenate/1171
  t10/20 -> concatenate/1172
  t10/21 -> concatenate/1173
  t10/22 -> concatenate/1174
  t10/23 -> concatenate/1175
  t10/24 -> concatenate/1176
  t10/25 -> concatenate/1177
  t10/26 -> concatenate/1178
  t10/27 -> concatenate/1179
  t10/28 -> concatenate/1180
  t10/29 -> concatenate/1181
  t10/30 -> concatenate/1182
  t10/31 -> concatenate/1183
  t10/32 -> concatenate/1184
  t10/33 -> concatenate/1185
  t10/34 -> concatenate/1186
  t10/35 -> concatenate/1187
  t10/36 -> concatenate/1188
  t10/37 -> concatenate/1189
  t10/38 -> concatenate/1190
  t10/39 -> concatenate/1191
  t10/40 -> concatenate/1192
  t10/41 -> concatenate/1193
  t10/42 -> concatenate/1194
  t10/43 -> concatenate/1195
  t10/44 -> concatenate/1196
  t10/45 -> concatenate/1197
  t10/46 -> concatenate/1198
  t10/47 -> concatenate/1199
  t10/48 -> concatenate/1200
  t10/49 -> concatenate/1201
  t10/50 -> concatenate/1202
  t10/51 -> concatenate/1203
  t10/52 -> concatenate/1204
  t10/53 -> concatenate/1205
  t10/54 -> concatenate/1206
  t10/55 -> concatenate/1207
  t10/56 -> concatenate/1208
  t10/57 -> concatenate/1209
  t10/58 -> concatenate/1210
  t10/59 -> concatenate/1211
  t10/60 -> concatenate/1212
  t10/61 -> concatenate/1213
  t10/62 -> concatenate/1214
  t10/63 -> concatenate/1215
  t10/64 -> concatenate/1216
  t10/65 -> concatenate/1217
  t10/66 -> concatenate/1218
  t10/67 -> concatenate/1219
  t10/68 -> concatenate/1220
  t10/69 -> concatenate/1221
  t10/70 -> concatenate/1222
  t10/71 -> concatenate/1223
  t10/72 -> concatenate/1224
  t10/73 -> concatenate/1225
  t10/74 -> concatenate/1226
  t10/75 -> concatenate/1227
  t10/76 -> concatenate/1228
  t10/77 -> concatenate/1229
  t10/78 -> concatenate/1230
  t10/79 -> concatenate/1231
  t10/80 -> concatenate/1232
  t10/81 -> concatenate/1233
  t10/82 -> concatenate/1234
  t10/83 -> concatenate/1235
  t10/84 -> concatenate/1236
  t10/85 -> concatenate/1237
  t10/86 -> concatenate/1238
  t10/87 -> concatenate/1239
  t10/88 -> concatenate/1240
  t10/89 -> concatenate/1241
  t10/90 -> concatenate/1242
  t10/91 -> concatenate/1243
  t10/92 -> concatenate/1244
  t10/93 -> concatenate/1245
  t10/94 -> concatenate/1246
  t10/95 -> concatenate/1247
  t10/96 -> concatenate/1248
  t10/97 -> concatenate/1249
  t10/98 -> concatenate/1250
  t10/99 -> concatenate/1251
  t10/100 -> concatenate/1252
  t10/101 -> concatenate/1253
  t10/102 -> concatenate/1254
  t10/103 -> concatenate/1255
  t10/104 -> concatenate/1256
  t10/105 -> concatenate/1257
  t10/106 -> concatenate/1258
  t10/107 -> concatenate/1259
  t10/108 -> concatenate/1260
  t10/109 -> concatenate/1261
  t10/110 -> concatenate/1262
  t10/111 -> concatenate/1263
  t10/112 -> concatenate/1264
  t10/113 -> concatenate/1265
  t10/114 -> concatenate/1266
  t10/115 -> concatenate/1267
  t10/116 -> concatenate/1268
  t10/117 -> concatenate/1269
  t10/118 -> concatenate/1270
  t10/119 -> concatenate/1271
  t10/120 -> concatenate/1272
  t10/121 -> concatenate/1273
  t10/122 -> concatenate/1274
  t10/123 -> concatenate/1275
  t10/124 -> concatenate/1276
  t10/125 -> concatenate/1277
  t10/126 -> concatenate/1278
  t10/127 -> concatenate/1279
  t10/128 -> concatenate/1280
  t11/1 -> concatenate/1281
  t11/2 -> concatenate/1282
  t11/3 -> concatenate/1283
  t11/4 -> concatenate/1284
  t11/5 -> concatenate/1285
  t11/6 -> concatenate/1286
  t11/7 -> concatenate/1287
  t11/8 -> concatenate/1288
  t11/9 -> concatenate/1289
  t11/10 -> concatenate/1290
  t11/11 -> concatenate/1291
  t11/12 -> concatenate/1292
  t11/13 -> concatenate/1293
  t11/14 -> concatenate/1294
  t11/15 -> concatenate/1295
  t11/16 -> concatenate/1296
  t11/17 -> concatenate/1297
  t11/18 -> concatenate/1298
  t11/19 -> concatenate/1299
  t11/20 -> concatenate/1300
  t11/21 -> concatenate/1301
  t11/22 -> concatenate/1302
  t11/23 -> concatenate/1303
  t11/24 -> concatenate/1304
  t11/25 -> concatenate/1305
  t11/26 -> concatenate/1306
  t11/27 -> concatenate/1307
  t11/28 -> concatenate/1308
  t11/29 -> concatenate/1309
  t11/30 -> concatenate/1310
  t11/31 -> concatenate/1311
  t11/32 -> concatenate/1312
  t11/33 -> concatenate/1313
  t11/34 -> concatenate/1314
  t11/35 -> concatenate/1315
  t11/36 -> concatenate/1316
  t11/37 -> concatenate/1317
  t11/38 -> concatenate/1318
  t11/39 -> concatenate/1319
  t11/40 -> concatenate/1320
  t11/41 -> concatenate/1321
  t11/42 -> concatenate/1322
  t11/43 -> concatenate/1323
  t11/44 -> concatenate/1324
  t11/45 -> concatenate/1325
  t11/46 -> concatenate/1326
  t11/47 -> concatenate/1327
  t11/48 -> concatenate/1328
  t11/49 -> concatenate/1329
  t11/50 -> concatenate/1330
  t11/51 -> concatenate/1331
  t11/52 -> concatenate/1332
  t11/53 -> concatenate/1333
  t11/54 -> concatenate/1334
  t11/55 -> concatenate/1335
  t11/56 -> concatenate/1336
  t11/57 -> concatenate/1337
  t11/58 -> concatenate/1338
  t11/59 -> concatenate/1339
  t11/60 -> concatenate/1340
  t11/61 -> concatenate/1341
  t11/62 -> concatenate/1342
  t11/63 -> concatenate/1343
  t11/64 -> concatenate/1344
  t11/65 -> concatenate/1345
  t11/66 -> concatenate/1346
  t11/67 -> concatenate/1347
  t11/68 -> concatenate/1348
  t11/69 -> concatenate/1349
  t11/70 -> concatenate/1350
  t11/71 -> concatenate/1351
  t11/72 -> concatenate/1352
  t11/73 -> concatenate/1353
  t11/74 -> concatenate/1354
  t11/75 -> concatenate/1355
  t11/76 -> concatenate/1356
  t11/77 -> concatenate/1357
  t11/78 -> concatenate/1358
  t11/79 -> concatenate/1359
  t11/80 -> concatenate/1360
  t11/81 -> concatenate/1361
  t11/82 -> concatenate/1362
  t11/83 -> concatenate/1363
  t11/84 -> concatenate/1364
  t11/85 -> concatenate/1365
  t11/86 -> concatenate/1366
  t11/87 -> concatenate/1367
  t11/88 -> concatenate/1368
  t11/89 -> concatenate/1369
  t11/90 -> concatenate/1370
  t11/91 -> concatenate/1371
  t11/92 -> concatenate/1372
  t11/93 -> concatenate/1373
  t11/94 -> concatenate/1374
  t11/95 -> concatenate/1375
  t11/96 -> concatenate/1376
  t11/97 -> concatenate/1377
  t11/98 -> concatenate/1378
  t11/99 -> concatenate/1379
  t11/100 -> concatenate/1380
  t11/101 -> concatenate/1381
  t11/102 -> concatenate/1382
  t11/103 -> concatenate/1383
  t11/104 -> concatenate/1384
  t11/105 -> concatenate/1385
  t11/106 -> concatenate/1386
  t11/107 -> concatenate/1387
  t11/108 -> concatenate/1388
  t11/109 -> concatenate/1389
  t11/110 -> concatenate/1390
  t11/111 -> concatenate/1391
  t11/112 -> concatenate/1392
  t11/113 -> concatenate/1393
  t11/114 -> concatenate/1394
  t11/115 -> concatenate/1395
  t11/116 -> concatenate/1396
  t11/117 -> concatenate/1397
  t11/118 -> concatenate/1398
  t11/119 -> concatenate/1399
  t11/120 -> concatenate/1400
  t11/121 -> concatenate/1401
  t11/122 -> concatenate/1402
  t11/123 -> concatenate/1403
  t11/124 -> concatenate/1404
  t11/125 -> concatenate/1405
  t11/126 -> concatenate/1406
  t11/127 -> concatenate/1407
  t11/128 -> concatenate/1408
  t12/1 -> concatenate/1409
  t12/2 -> concatenate/1410
  t12/3 -> concatenate/1411
  t12/4 -> concatenate/1412
  t12/5 -> concatenate/1413
  t12/6 -> concatenate/1414
  t12/7 -> concatenate/1415
  t12/8 -> concatenate/1416
  t12/9 -> concatenate/1417
  t12/10 -> concatenate/1418
  t12/11 -> concatenate/1419
  t12/12 -> concatenate/1420
  t12/13 -> concatenate/1421
  t12/14 -> concatenate/1422
  t12/15 -> concatenate/1423
  t12/16 -> concatenate/1424
  t12/17 -> concatenate/1425
  t12/18 -> concatenate/1426
  t12/19 -> concatenate/1427
  t12/20 -> concatenate/1428
  t12/21 -> concatenate/1429
  t12/22 -> concatenate/1430
  t12/23 -> concatenate/1431
  t12/24 -> concatenate/1432
  t12/25 -> concatenate/1433
  t12/26 -> concatenate/1434
  t12/27 -> concatenate/1435
  t12/28 -> concatenate/1436
  t12/29 -> concatenate/1437
  t12/30 -> concatenate/1438
  t12/31 -> concatenate/1439
  t12/32 -> concatenate/1440
  t12/33 -> concatenate/1441
  t12/34 -> concatenate/1442
  t12/35 -> concatenate/1443
  t12/36 -> concatenate/1444
  t12/37 -> concatenate/1445
  t12/38 -> concatenate/1446
  t12/39 -> concatenate/1447
  t12/40 -> concatenate/1448
  t12/41 -> concatenate/1449
  t12/42 -> concatenate/1450
  t12/43 -> concatenate/1451
  t12/44 -> concatenate/1452
  t12/45 -> concatenate/1453
  t12/46 -> concatenate/1454
  t12/47 -> concatenate/1455
  t12/48 -> concatenate/1456
  t12/49 -> concatenate/1457
  t12/50 -> concatenate/1458
  t12/51 -> concatenate/1459
  t12/52 -> concatenate/1460
  t12/53 -> concatenate/1461
  t12/54 -> concatenate/1462
  t12/55 -> concatenate/1463
  t12/56 -> concatenate/1464
  t12/57 -> concatenate/1465
  t12/58 -> concatenate/1466
  t12/59 -> concatenate/1467
  t12/60 -> concatenate/1468
  t12/61 -> concatenate/1469
  t12/62 -> concatenate/1470
  t12/63 -> concatenate/1471
  t12/64 -> concatenate/1472
  t12/65 -> concatenate/1473
  t12/66 -> concatenate/1474
  t12/67 -> concatenate/1475
  t12/68 -> concatenate/1476
  t12/69 -> concatenate/1477
  t12/70 -> concatenate/1478
  t12/71 -> concatenate/1479
  t12/72 -> concatenate/1480
  t12/73 -> concatenate/1481
  t12/74 -> concatenate/1482
  t12/75 -> concatenate/1483
  t12/76 -> concatenate/1484
  t12/77 -> concatenate/1485
  t12/78 -> concatenate/1486
  t12/79 -> concatenate/1487
  t12/80 -> concatenate/1488
  t12/81 -> concatenate/1489
  t12/82 -> concatenate/1490
  t12/83 -> concatenate/1491
  t12/84 -> concatenate/1492
  t12/85 -> concatenate/1493
  t12/86 -> concatenate/1494
  t12/87 -> concatenate/1495
  t12/88 -> concatenate/1496
  t12/89 -> concatenate/1497
  t12/90 -> concatenate/1498
  t12/91 -> concatenate/1499
  t12/92 -> concatenate/1500
  t12/93 -> concatenate/1501
  t12/94 -> concatenate/1502
  t12/95 -> concatenate/1503
  t12/96 -> concatenate/1504
  t12/97 -> concatenate/1505
  t12/98 -> concatenate/1506
  t12/99 -> concatenate/1507
  t12/100 -> concatenate/1508
  t12/101 -> concatenate/1509
  t12/102 -> concatenate/1510
  t12/103 -> concatenate/1511
  t12/104 -> concatenate/1512
  t12/105 -> concatenate/1513
  t12/106 -> concatenate/1514
  t12/107 -> concatenate/1515
  t12/108 -> concatenate/1516
  t12/109 -> concatenate/1517
  t12/110 -> concatenate/1518
  t12/111 -> concatenate/1519
  t12/112 -> concatenate/1520
  t12/113 -> concatenate/1521
  t12/114 -> concatenate/1522
  t12/115 -> concatenate/1523
  t12/116 -> concatenate/1524
  t12/117 -> concatenate/1525
  t12/118 -> concatenate/1526
  t12/119 -> concatenate/1527
  t12/120 -> concatenate/1528
  t12/121 -> concatenate/1529
  t12/122 -> concatenate/1530
  t12/123 -> concatenate/1531
  t12/124 -> concatenate/1532
  t12/125 -> concatenate/1533
  t12/126 -> concatenate/1534
  t12/127 -> concatenate/1535
  t12/128 -> concatenate/1536
  t13/1 -> concatenate/1537
  t13/2 -> concatenate/1538
  t13/3 -> concatenate/1539
  t13/4 -> concatenate/1540
  t13/5 -> concatenate/1541
  t13/6 -> concatenate/1542
  t13/7 -> concatenate/1543
  t13/8 -> concatenate/1544
  t13/9 -> concatenate/1545
  t13/10 -> concatenate/1546
  t13/11 -> concatenate/1547
  t13/12 -> concatenate/1548
  t13/13 -> concatenate/1549
  t13/14 -> concatenate/1550
  t13/15 -> concatenate/1551
  t13/16 -> concatenate/1552
  t13/17 -> concatenate/1553
  t13/18 -> concatenate/1554
  t13/19 -> concatenate/1555
  t13/20 -> concatenate/1556
  t13/21 -> concatenate/1557
  t13/22 -> concatenate/1558
  t13/23 -> concatenate/1559
  t13/24 -> concatenate/1560
  t13/25 -> concatenate/1561
  t13/26 -> concatenate/1562
  t13/27 -> concatenate/1563
  t13/28 -> concatenate/1564
  t13/29 -> concatenate/1565
  t13/30 -> concatenate/1566
  t13/31 -> concatenate/1567
  t13/32 -> concatenate/1568
  t13/33 -> concatenate/1569
  t13/34 -> concatenate/1570
  t13/35 -> concatenate/1571
  t13/36 -> concatenate/1572
  t13/37 -> concatenate/1573
  t13/38 -> concatenate/1574
  t13/39 -> concatenate/1575
  t13/40 -> concatenate/1576
  t13/41 -> concatenate/1577
  t13/42 -> concatenate/1578
  t13/43 -> concatenate/1579
  t13/44 -> concatenate/1580
  t13/45 -> concatenate/1581
  t13/46 -> concatenate/1582
  t13/47 -> concatenate/1583
  t13/48 -> concatenate/1584
  t13/49 -> concatenate/1585
  t13/50 -> concatenate/1586
  t13/51 -> concatenate/1587
  t13/52 -> concatenate/1588
  t13/53 -> concatenate/1589
  t13/54 -> concatenate/1590
  t13/55 -> concatenate/1591
  t13/56 -> concatenate/1592
  t13/57 -> concatenate/1593
  t13/58 -> concatenate/1594
  t13/59 -> concatenate/1595
  t13/60 -> concatenate/1596
  t13/61 -> concatenate/1597
  t13/62 -> concatenate/1598
  t13/63 -> concatenate/1599
  t13/64 -> concatenate/1600
  t13/65 -> concatenate/1601
  t13/66 -> concatenate/1602
  t13/67 -> concatenate/1603
  t13/68 -> concatenate/1604
  t13/69 -> concatenate/1605
  t13/70 -> concatenate/1606
  t13/71 -> concatenate/1607
  t13/72 -> concatenate/1608
  t13/73 -> concatenate/1609
  t13/74 -> concatenate/1610
  t13/75 -> concatenate/1611
  t13/76 -> concatenate/1612
  t13/77 -> concatenate/1613
  t13/78 -> concatenate/1614
  t13/79 -> concatenate/1615
  t13/80 -> concatenate/1616
  t13/81 -> concatenate/1617
  t13/82 -> concatenate/1618
  t13/83 -> concatenate/1619
  t13/84 -> concatenate/1620
  t13/85 -> concatenate/1621
  t13/86 -> concatenate/1622
  t13/87 -> concatenate/1623
  t13/88 -> concatenate/1624
  t13/89 -> concatenate/1625
  t13/90 -> concatenate/1626
  t13/91 -> concatenate/1627
  t13/92 -> concatenate/1628
  t13/93 -> concatenate/1629
  t13/94 -> concatenate/1630
  t13/95 -> concatenate/1631
  t13/96 -> concatenate/1632
  t13/97 -> concatenate/1633
  t13/98 -> concatenate/1634
  t13/99 -> concatenate/1635
  t13/100 -> concatenate/1636
  t13/101 -> concatenate/1637
  t13/102 -> concatenate/1638
  t13/103 -> concatenate/1639
  t13/104 -> concatenate/1640
  t13/105 -> concatenate/1641
  t13/106 -> concatenate/1642
  t13/107 -> concatenate/1643
  t13/108 -> concatenate/1644
  t13/109 -> concatenate/1645
  t13/110 -> concatenate/1646
  t13/111 -> concatenate/1647
  t13/112 -> concatenate/1648
  t13/113 -> concatenate/1649
  t13/114 -> concatenate/1650
  t13/115 -> concatenate/1651
  t13/116 -> concatenate/1652
  t13/117 -> concatenate/1653
  t13/118 -> concatenate/1654
  t13/119 -> concatenate/1655
  t13/120 -> concatenate/1656
  t13/121 -> concatenate/1657
  t13/122 -> concatenate/1658
  t13/123 -> concatenate/1659
  t13/124 -> concatenate/1660
  t13/125 -> concatenate/1661
  t13/126 -> concatenate/1662
  t13/127 -> concatenate/1663
  t13/128 -> concatenate/1664
  t14/1 -> concatenate/1665
  t14/2 -> concatenate/1666
  t14/3 -> concatenate/1667
  t14/4 -> concatenate/1668
  t14/5 -> concatenate/1669
  t14/6 -> concatenate/1670
  t14/7 -> concatenate/1671
  t14/8 -> concatenate/1672
  t14/9 -> concatenate/1673
  t14/10 -> concatenate/1674
  t14/11 -> concatenate/1675
  t14/12 -> concatenate/1676
  t14/13 -> concatenate/1677
  t14/14 -> concatenate/1678
  t14/15 -> concatenate/1679
  t14/16 -> concatenate/1680
  t14/17 -> concatenate/1681
  t14/18 -> concatenate/1682
  t14/19 -> concatenate/1683
  t14/20 -> concatenate/1684
  t14/21 -> concatenate/1685
  t14/22 -> concatenate/1686
  t14/23 -> concatenate/1687
  t14/24 -> concatenate/1688
  t14/25 -> concatenate/1689
  t14/26 -> concatenate/1690
  t14/27 -> concatenate/1691
  t14/28 -> concatenate/1692
  t14/29 -> concatenate/1693
  t14/30 -> concatenate/1694
  t14/31 -> concatenate/1695
  t14/32 -> concatenate/1696
  t14/33 -> concatenate/1697
  t14/34 -> concatenate/1698
  t14/35 -> concatenate/1699
  t14/36 -> concatenate/1700
  t14/37 -> concatenate/1701
  t14/38 -> concatenate/1702
  t14/39 -> concatenate/1703
  t14/40 -> concatenate/1704
  t14/41 -> concatenate/1705
  t14/42 -> concatenate/1706
  t14/43 -> concatenate/1707
  t14/44 -> concatenate/1708
  t14/45 -> concatenate/1709
  t14/46 -> concatenate/1710
  t14/47 -> concatenate/1711
  t14/48 -> concatenate/1712
  t14/49 -> concatenate/1713
  t14/50 -> concatenate/1714
  t14/51 -> concatenate/1715
  t14/52 -> concatenate/1716
  t14/53 -> concatenate/1717
  t14/54 -> concatenate/1718
  t14/55 -> concatenate/1719
  t14/56 -> concatenate/1720
  t14/57 -> concatenate/1721
  t14/58 -> concatenate/1722
  t14/59 -> concatenate/1723
  t14/60 -> concatenate/1724
  t14/61 -> concatenate/1725
  t14/62 -> concatenate/1726
  t14/63 -> concatenate/1727
  t14/64 -> concatenate/1728
  t14/65 -> concatenate/1729
  t14/66 -> concatenate/1730
  t14/67 -> concatenate/1731
  t14/68 -> concatenate/1732
  t14/69 -> concatenate/1733
  t14/70 -> concatenate/1734
  t14/71 -> concatenate/1735
  t14/72 -> concatenate/1736
  t14/73 -> concatenate/1737
  t14/74 -> concatenate/1738
  t14/75 -> concatenate/1739
  t14/76 -> concatenate/1740
  t14/77 -> concatenate/1741
  t14/78 -> concatenate/1742
  t14/79 -> concatenate/1743
  t14/80 -> concatenate/1744
  t14/81 -> concatenate/1745
  t14/82 -> concatenate/1746
  t14/83 -> concatenate/1747
  t14/84 -> concatenate/1748
  t14/85 -> concatenate/1749
  t14/86 -> concatenate/1750
  t14/87 -> concatenate/1751
  t14/88 -> concatenate/1752
  t14/89 -> concatenate/1753
  t14/90 -> concatenate/1754
  t14/91 -> concatenate/1755
  t14/92 -> concatenate/1756
  t14/93 -> concatenate/1757
  t14/94 -> concatenate/1758
  t14/95 -> concatenate/1759
  t14/96 -> concatenate/1760
  t14/97 -> concatenate/1761
  t14/98 -> concatenate/1762
  t14/99 -> concatenate/1763
  t14/100 -> concatenate/1764
  t14/101 -> concatenate/1765
  t14/102 -> concatenate/1766
  t14/103 -> concatenate/1767
  t14/104 -> concatenate/1768
  t14/105 -> concatenate/1769
  t14/106 -> concatenate/1770
  t14/107 -> concatenate/1771
  t14/108 -> concatenate/1772
  t14/109 -> concatenate/1773
  t14/110 -> concatenate/1774
  t14/111 -> concatenate/1775
  t14/112 -> concatenate/1776
  t14/113 -> concatenate/1777
  t14/114 -> concatenate/1778
  t14/115 -> concatenate/1779
  t14/116 -> concatenate/1780
  t14/117 -> concatenate/1781
  t14/118 -> concatenate/1782
  t14/119 -> concatenate/1783
  t14/120 -> concatenate/1784
  t14/121 -> concatenate/1785
  t14/122 -> concatenate/1786
  t14/123 -> concatenate/1787
  t14/124 -> concatenate/1788
  t14/125 -> concatenate/1789
  t14/126 -> concatenate/1790
  t14/127 -> concatenate/1791
  t14/128 -> concatenate/1792
  t15/1 -> concatenate/1793
  t15/2 -> concatenate/1794
  t15/3 -> concatenate/1795
  t15/4 -> concatenate/1796
  t15/5 -> concatenate/1797
  t15/6 -> concatenate/1798
  t15/7 -> concatenate/1799
  t15/8 -> concatenate/1800
  t15/9 -> concatenate/1801
  t15/10 -> concatenate/1802
  t15/11 -> concatenate/1803
  t15/12 -> concatenate/1804
  t15/13 -> concatenate/1805
  t15/14 -> concatenate/1806
  t15/15 -> concatenate/1807
  t15/16 -> concatenate/1808
  t15/17 -> concatenate/1809
  t15/18 -> concatenate/1810
  t15/19 -> concatenate/1811
  t15/20 -> concatenate/1812
  t15/21 -> concatenate/1813
  t15/22 -> concatenate/1814
  t15/23 -> concatenate/1815
  t15/24 -> concatenate/1816
  t15/25 -> concatenate/1817
  t15/26 -> concatenate/1818
  t15/27 -> concatenate/1819
  t15/28 -> concatenate/1820
  t15/29 -> concatenate/1821
  t15/30 -> concatenate/1822
  t15/31 -> concatenate/1823
  t15/32 -> concatenate/1824
  t15/33 -> concatenate/1825
  t15/34 -> concatenate/1826
  t15/35 -> concatenate/1827
  t15/36 -> concatenate/1828
  t15/37 -> concatenate/1829
  t15/38 -> concatenate/1830
  t15/39 -> concatenate/1831
  t15/40 -> concatenate/1832
  t15/41 -> concatenate/1833
  t15/42 -> concatenate/1834
  t15/43 -> concatenate/1835
  t15/44 -> concatenate/1836
  t15/45 -> concatenate/1837
  t15/46 -> concatenate/1838
  t15/47 -> concatenate/1839
  t15/48 -> concatenate/1840
  t15/49 -> concatenate/1841
  t15/50 -> concatenate/1842
  t15/51 -> concatenate/1843
  t15/52 -> concatenate/1844
  t15/53 -> concatenate/1845
  t15/54 -> concatenate/1846
  t15/55 -> concatenate/1847
  t15/56 -> concatenate/1848
  t15/57 -> concatenate/1849
  t15/58 -> concatenate/1850
  t15/59 -> concatenate/1851
  t15/60 -> concatenate/1852
  t15/61 -> concatenate/1853
  t15/62 -> concatenate/1854
  t15/63 -> concatenate/1855
  t15/64 -> concatenate/1856
  t15/65 -> concatenate/1857
  t15/66 -> concatenate/1858
  t15/67 -> concatenate/1859
  t15/68 -> concatenate/1860
  t15/69 -> concatenate/1861
  t15/70 -> concatenate/1862
  t15/71 -> concatenate/1863
  t15/72 -> concatenate/1864
  t15/73 -> concatenate/1865
  t15/74 -> concatenate/1866
  t15/75 -> concatenate/1867
  t15/76 -> concatenate/1868
  t15/77 -> concatenate/1869
  t15/78 -> concatenate/1870
  t15/79 -> concatenate/1871
  t15/80 -> concatenate/1872
  t15/81 -> concatenate/1873
  t15/82 -> concatenate/1874
  t15/83 -> concatenate/1875
  t15/84 -> concatenate/1876
  t15/85 -> concatenate/1877
  t15/86 -> concatenate/1878
  t15/87 -> concatenate/1879
  t15/88 -> concatenate/1880
  t15/89 -> concatenate/1881
  t15/90 -> concatenate/1882
  t15/91 -> concatenate/1883
  t15/92 -> concatenate/1884
  t15/93 -> concatenate/1885
  t15/94 -> concatenate/1886
  t15/95 -> concatenate/1887
  t15/96 -> concatenate/1888
  t15/97 -> concatenate/1889
  t15/98 -> concatenate/1890
  t15/99 -> concatenate/1891
  t15/100 -> concatenate/1892
  t15/101 -> concatenate/1893
  t15/102 -> concatenate/1894
  t15/103 -> concatenate/1895
  t15/104 -> concatenate/1896
  t15/105 -> concatenate/1897
  t15/106 -> concatenate/1898
  t15/107 -> concatenate/1899
  t15/108 -> concatenate/1900
  t15/109 -> concatenate/1901
  t15/110 -> concatenate/1902
  t15/111 -> concatenate/1903
  t15/112 -> concatenate/1904
  t15/113 -> concatenate/1905
  t15/114 -> concatenate/1906
  t15/115 -> concatenate/1907
  t15/116 -> concatenate/1908
  t15/117 -> concatenate/1909
  t15/118 -> concatenate/1910
  t15/119 -> concatenate/1911
  t15/120 -> concatenate/1912
  t15/121 -> concatenate/1913
  t15/122 -> concatenate/1914
  t15/123 -> concatenate/1915
  t15/124 -> concatenate/1916
  t15/125 -> concatenate/1917
  t15/126 -> concatenate/1918
  t15/127 -> concatenate/1919
  t15/128 -> concatenate/1920
  t16/1 -> concatenate/1921
  t16/2 -> concatenate/1922
  t16/3 -> concatenate/1923
  t16/4 -> concatenate/1924
  t16/5 -> concatenate/1925
  t16/6 -> concatenate/1926
  t16/7 -> concatenate/1927
  t16/8 -> concatenate/1928
  t16/9 -> concatenate/1929
  t16/10 -> concatenate/1930
  t16/11 -> concatenate/1931
  t16/12 -> concatenate/1932
  t16/13 -> concatenate/1933
  t16/14 -> concatenate/1934
  t16/15 -> concatenate/1935
  t16/16 -> concatenate/1936
  t16/17 -> concatenate/1937
  t16/18 -> concatenate/1938
  t16/19 -> concatenate/1939
  t16/20 -> concatenate/1940
  t16/21 -> concatenate/1941
  t16/22 -> concatenate/1942
  t16/23 -> concatenate/1943
  t16/24 -> concatenate/1944
  t16/25 -> concatenate/1945
  t16/26 -> concatenate/1946
  t16/27 -> concatenate/1947
  t16/28 -> concatenate/1948
  t16/29 -> concatenate/1949
  t16/30 -> concatenate/1950
  t16/31 -> concatenate/1951
  t16/32 -> concatenate/1952
  t16/33 -> concatenate/1953
  t16/34 -> concatenate/1954
  t16/35 -> concatenate/1955
  t16/36 -> concatenate/1956
  t16/37 -> concatenate/1957
  t16/38 -> concatenate/1958
  t16/39 -> concatenate/1959
  t16/40 -> concatenate/1960
  t16/41 -> concatenate/1961
  t16/42 -> concatenate/1962
  t16/43 -> concatenate/1963
  t16/44 -> concatenate/1964
  t16/45 -> concatenate/1965
  t16/46 -> concatenate/1966
  t16/47 -> concatenate/1967
  t16/48 -> concatenate/1968
  t16/49 -> concatenate/1969
  t16/50 -> concatenate/1970
  t16/51 -> concatenate/1971
  t16/52 -> concatenate/1972
  t16/53 -> concatenate/1973
  t16/54 -> concatenate/1974
  t16/55 -> concatenate/1975
  t16/56 -> concatenate/1976
  t16/57 -> concatenate/1977
  t16/58 -> concatenate/1978
  t16/59 -> concatenate/1979
  t16/60 -> concatenate/1980
  t16/61 -> concatenate/1981
  t16/62 -> concatenate/1982
  t16/63 -> concatenate/1983
  t16/64 -> concatenate/1984
  t16/65 -> concatenate/1985
  t16/66 -> concatenate/1986
  t16/67 -> concatenate/1987
  t16/68 -> concatenate/1988
  t16/69 -> concatenate/1989
  t16/70 -> concatenate/1990
  t16/71 -> concatenate/1991
  t16/72 -> concatenate/1992
  t16/73 -> concatenate/1993
  t16/74 -> concatenate/1994
  t16/75 -> concatenate/1995
  t16/76 -> concatenate/1996
  t16/77 -> concatenate/1997
  t16/78 -> concatenate/1998
  t16/79 -> concatenate/1999
  t16/80 -> concatenate/2000
  t16/81 -> concatenate/2001
  t16/82 -> concatenate/2002
  t16/83 -> concatenate/2003
  t16/84 -> concatenate/2004
  t16/85 -> concatenate/2005
  t16/86 -> concatenate/2006
  t16/87 -> concatenate/2007
  t16/88 -> concatenate/2008
  t16/89 -> concatenate/2009
  t16/90 -> concatenate/2010
  t16/91 -> concatenate/2011
  t16/92 -> concatenate/2012
  t16/93 -> concatenate/2013
  t16/94 -> concatenate/2014
  t16/95 -> concatenate/2015
  t16/96 -> concatenate/2016
  t16/97 -> concatenate/2017
  t16/98 -> concatenate/2018
  t16/99 -> concatenate/2019
  t16/100 -> concatenate/2020
  t16/101 -> concatenate/2021
  t16/102 -> concatenate/2022
  t16/103 -> concatenate/2023
  t16/104 -> concatenate/2024
  t16/105 -> concatenate/2025
  t16/106 -> concatenate/2026
  t16/107 -> concatenate/2027
  t16/108 -> concatenate/2028
  t16/109 -> concatenate/2029
  t16/110 -> concatenate/2030
  t16/111 -> concatenate/2031
  t16/112 -> concatenate/2032
  t16/113 -> concatenate/2033
  t16/114 -> concatenate/2034
  t16/115 -> concatenate/2035
  t16/116 -> concatenate/2036
  t16/117 -> concatenate/2037
  t16/118 -> concatenate/2038
  t16/119 -> concatenate/2039
  t16/120 -> concatenate/2040
  t16/121 -> concatenate/2041
  t16/122 -> concatenate/2042
  t16/123 -> concatenate/2043
  t16/124 -> concatenate/2044
  t16/125 -> concatenate/2045
  t16/126 -> concatenate/2046
  t16/127 -> concatenate/2047
  t16/128 -> concatenate/2048
  t17/1 -> concatenate/2049
  t17/2 -> concatenate/2050
  t17/3 -> concatenate/2051
  t17/4 -> concatenate/2052
  t17/5 -> concatenate/2053
  t17/6 -> concatenate/2054
  t17/7 -> concatenate/2055
  t17/8 -> concatenate/2056
  t17/9 -> concatenate/2057
  t17/10 -> concatenate/2058
  t17/11 -> concatenate/2059
  t17/12 -> concatenate/2060
  t17/13 -> concatenate/2061
  t17/14 -> concatenate/2062
  t17/15 -> concatenate/2063
  t17/16 -> concatenate/2064
  t17/17 -> concatenate/2065
  t17/18 -> concatenate/2066
  t17/19 -> concatenate/2067
  t17/20 -> concatenate/2068
  t17/21 -> concatenate/2069
  t17/22 -> concatenate/2070
  t17/23 -> concatenate/2071
  t17/24 -> concatenate/2072
  t17/25 -> concatenate/2073
  t17/26 -> concatenate/2074
  t17/27 -> concatenate/2075
  t17/28 -> concatenate/2076
  t17/29 -> concatenate/2077
  t17/30 -> concatenate/2078
  t17/31 -> concatenate/2079
  t17/32 -> concatenate/2080
  t17/33 -> concatenate/2081
  t17/34 -> concatenate/2082
  t17/35 -> concatenate/2083
  t17/36 -> concatenate/2084
  t17/37 -> concatenate/2085
  t17/38 -> concatenate/2086
  t17/39 -> concatenate/2087
  t17/40 -> concatenate/2088
  t17/41 -> concatenate/2089
  t17/42 -> concatenate/2090
  t17/43 -> concatenate/2091
  t17/44 -> concatenate/2092
  t17/45 -> concatenate/2093
  t17/46 -> concatenate/2094
  t17/47 -> concatenate/2095
  t17/48 -> concatenate/2096
  t17/49 -> concatenate/2097
  t17/50 -> concatenate/2098
  t17/51 -> concatenate/2099
  t17/52 -> concatenate/2100
  t17/53 -> concatenate/2101
  t17/54 -> concatenate/2102
  t17/55 -> concatenate/2103
  t17/56 -> concatenate/2104
  t17/57 -> concatenate/2105
  t17/58 -> concatenate/2106
  t17/59 -> concatenate/2107
  t17/60 -> concatenate/2108
  t17/61 -> concatenate/2109
  t17/62 -> concatenate/2110
  t17/63 -> concatenate/2111
  t17/64 -> concatenate/2112
  t17/65 -> concatenate/2113
  t17/66 -> concatenate/2114
  t17/67 -> concatenate/2115
  t17/68 -> concatenate/2116
  t17/69 -> concatenate/2117
  t17/70 -> concatenate/2118
  t17/71 -> concatenate/2119
  t17/72 -> concatenate/2120
  t17/73 -> concatenate/2121
  t17/74 -> concatenate/2122
  t17/75 -> concatenate/2123
  t17/76 -> concatenate/2124
  t17/77 -> concatenate/2125
  t17/78 -> concatenate/2126
  t17/79 -> concatenate/2127
  t17/80 -> concatenate/2128
  t17/81 -> concatenate/2129
  t17/82 -> concatenate/2130
  t17/83 -> concatenate/2131
  t17/84 -> concatenate/2132
  t17/85 -> concatenate/2133
  t17/86 -> concatenate/2134
  t17/87 -> concatenate/2135
  t17/88 -> concatenate/2136
  t17/89 -> concatenate/2137
  t17/90 -> concatenate/2138
  t17/91 -> concatenate/2139
  t17/92 -> concatenate/2140
  t17/93 -> concatenate/2141
  t17/94 -> concatenate/2142
  t17/95 -> concatenate/2143
  t17/96 -> concatenate/2144
  t17/97 -> concatenate/2145
  t17/98 -> concatenate/2146
  t17/99 -> concatenate/2147
  t17/100 -> concatenate/2148
  t17/101 -> concatenate/2149
  t17/102 -> concatenate/2150
  t17/103 -> concatenate/2151
  t17/104 -> concatenate/2152
  t17/105 -> concatenate/2153
  t17/106 -> concatenate/2154
  t17/107 -> concatenate/2155
  t17/108 -> concatenate/2156
  t17/109 -> concatenate/2157
  t17/110 -> concatenate/2158
  t17/111 -> concatenate/2159
  t17/112 -> concatenate/2160
  t17/113 -> concatenate/2161
  t17/114 -> concatenate/2162
  t17/115 -> concatenate/2163
  t17/116 -> concatenate/2164
  t17/117 -> concatenate/2165
  t17/118 -> concatenate/2166
  t17/119 -> concatenate/2167
  t17/120 -> concatenate/2168
  t17/121 -> concatenate/2169
  t17/122 -> concatenate/2170
  t17/123 -> concatenate/2171
  t17/124 -> concatenate/2172
  t17/125 -> concatenate/2173
  t17/126 -> concatenate/2174
  t17/127 -> concatenate/2175
  t17/128 -> concatenate/2176
  t18/1 -> concatenate/2177
  t18/2 -> concatenate/2178
  t18/3 -> concatenate/2179
  t18/4 -> concatenate/2180
  t18/5 -> concatenate/2181
  t18/6 -> concatenate/2182
  t18/7 -> concatenate/2183
  t18/8 -> concatenate/2184
  t18/9 -> concatenate/2185
  t18/10 -> concatenate/2186
  t18/11 -> concatenate/2187
  t18/12 -> concatenate/2188
  t18/13 -> concatenate/2189
  t18/14 -> concatenate/2190
  t18/15 -> concatenate/2191
  t18/16 -> concatenate/2192
  t18/17 -> concatenate/2193
  t18/18 -> concatenate/2194
  t18/19 -> concatenate/2195
  t18/20 -> concatenate/2196
  t18/21 -> concatenate/2197
  t18/22 -> concatenate/2198
  t18/23 -> concatenate/2199
  t18/24 -> concatenate/2200
  t18/25 -> concatenate/2201
  t18/26 -> concatenate/2202
  t18/27 -> concatenate/2203
  t18/28 -> concatenate/2204
  t18/29 -> concatenate/2205
  t18/30 -> concatenate/2206
  t18/31 -> concatenate/2207
  t18/32 -> concatenate/2208
  t18/33 -> concatenate/2209
  t18/34 -> concatenate/2210
  t18/35 -> concatenate/2211
  t18/36 -> concatenate/2212
  t18/37 -> concatenate/2213
  t18/38 -> concatenate/2214
  t18/39 -> concatenate/2215
  t18/40 -> concatenate/2216
  t18/41 -> concatenate/2217
  t18/42 -> concatenate/2218
  t18/43 -> concatenate/2219
  t18/44 -> concatenate/2220
  t18/45 -> concatenate/2221
  t18/46 -> concatenate/2222
  t18/47 -> concatenate/2223
  t18/48 -> concatenate/2224
  t18/49 -> concatenate/2225
  t18/50 -> concatenate/2226
  t18/51 -> concatenate/2227
  t18/52 -> concatenate/2228
  t18/53 -> concatenate/2229
  t18/54 -> concatenate/2230
  t18/55 -> concatenate/2231
  t18/56 -> concatenate/2232
  t18/57 -> concatenate/2233
  t18/58 -> concatenate/2234
  t18/59 -> concatenate/2235
  t18/60 -> concatenate/2236
  t18/61 -> concatenate/2237
  t18/62 -> concatenate/2238
  t18/63 -> concatenate/2239
  t18/64 -> concatenate/2240
  t18/65 -> concatenate/2241
  t18/66 -> concatenate/2242
  t18/67 -> concatenate/2243
  t18/68 -> concatenate/2244
  t18/69 -> concatenate/2245
  t18/70 -> concatenate/2246
  t18/71 -> concatenate/2247
  t18/72 -> concatenate/2248
  t18/73 -> concatenate/2249
  t18/74 -> concatenate/2250
  t18/75 -> concatenate/2251
  t18/76 -> concatenate/2252
  t18/77 -> concatenate/2253
  t18/78 -> concatenate/2254
  t18/79 -> concatenate/2255
  t18/80 -> concatenate/2256
  t18/81 -> concatenate/2257
  t18/82 -> concatenate/2258
  t18/83 -> concatenate/2259
  t18/84 -> concatenate/2260
  t18/85 -> concatenate/2261
  t18/86 -> concatenate/2262
  t18/87 -> concatenate/2263
  t18/88 -> concatenate/2264
  t18/89 -> concatenate/2265
  t18/90 -> concatenate/2266
  t18/91 -> concatenate/2267
  t18/92 -> concatenate/2268
  t18/93 -> concatenate/2269
  t18/94 -> concatenate/2270
  t18/95 -> concatenate/2271
  t18/96 -> concatenate/2272
  t18/97 -> concatenate/2273
  t18/98 -> concatenate/2274
  t18/99 -> concatenate/2275
  t18/100 -> concatenate/2276
  t18/101 -> concatenate/2277
  t18/102 -> concatenate/2278
  t18/103 -> concatenate/2279
  t18/104 -> concatenate/2280
  t18/105 -> concatenate/2281
  t18/106 -> concatenate/2282
  t18/107 -> concatenate/2283
  t18/108 -> concatenate/2284
  t18/109 -> concatenate/2285
  t18/110 -> concatenate/2286
  t18/111 -> concatenate/2287
  t18/112 -> concatenate/2288
  t18/113 -> concatenate/2289
  t18/114 -> concatenate/2290
  t18/115 -> concatenate/2291
  t18/116 -> concatenate/2292
  t18/117 -> concatenate/2293
  t18/118 -> concatenate/2294
  t18/119 -> concatenate/2295
  t18/120 -> concatenate/2296
  t18/121 -> concatenate/2297
  t18/122 -> concatenate/2298
  t18/123 -> concatenate/2299
  t18/124 -> concatenate/2300
  t18/125 -> concatenate/2301
  t18/126 -> concatenate/2302
  t18/127 -> concatenate/2303
  t18/128 -> concatenate/2304
  t19/1 -> concatenate/2305
  t19/2 -> concatenate/2306
  t19/3 -> concatenate/2307
  t19/4 -> concatenate/2308
  t19/5 -> concatenate/2309
  t19/6 -> concatenate/2310
  t19/7 -> concatenate/2311
  t19/8 -> concatenate/2312
  t19/9 -> concatenate/2313
  t19/10 -> concatenate/2314
  t19/11 -> concatenate/2315
  t19/12 -> concatenate/2316
  t19/13 -> concatenate/2317
  t19/14 -> concatenate/2318
  t19/15 -> concatenate/2319
  t19/16 -> concatenate/2320
  t19/17 -> concatenate/2321
  t19/18 -> concatenate/2322
  t19/19 -> concatenate/2323
  t19/20 -> concatenate/2324
  t19/21 -> concatenate/2325
  t19/22 -> concatenate/2326
  t19/23 -> concatenate/2327
  t19/24 -> concatenate/2328
  t19/25 -> concatenate/2329
  t19/26 -> concatenate/2330
  t19/27 -> concatenate/2331
  t19/28 -> concatenate/2332
  t19/29 -> concatenate/2333
  t19/30 -> concatenate/2334
  t19/31 -> concatenate/2335
  t19/32 -> concatenate/2336
  t19/33 -> concatenate/2337
  t19/34 -> concatenate/2338
  t19/35 -> concatenate/2339
  t19/36 -> concatenate/2340
  t19/37 -> concatenate/2341
  t19/38 -> concatenate/2342
  t19/39 -> concatenate/2343
  t19/40 -> concatenate/2344
  t19/41 -> concatenate/2345
  t19/42 -> concatenate/2346
  t19/43 -> concatenate/2347
  t19/44 -> concatenate/2348
  t19/45 -> concatenate/2349
  t19/46 -> concatenate/2350
  t19/47 -> concatenate/2351
  t19/48 -> concatenate/2352
  t19/49 -> concatenate/2353
  t19/50 -> concatenate/2354
  t19/51 -> concatenate/2355
  t19/52 -> concatenate/2356
  t19/53 -> concatenate/2357
  t19/54 -> concatenate/2358
  t19/55 -> concatenate/2359
  t19/56 -> concatenate/2360
  t19/57 -> concatenate/2361
  t19/58 -> concatenate/2362
  t19/59 -> concatenate/2363
  t19/60 -> concatenate/2364
  t19/61 -> concatenate/2365
  t19/62 -> concatenate/2366
  t19/63 -> concatenate/2367
  t19/64 -> concatenate/2368
  t19/65 -> concatenate/2369
  t19/66 -> concatenate/2370
  t19/67 -> concatenate/2371
  t19/68 -> concatenate/2372
  t19/69 -> concatenate/2373
  t19/70 -> concatenate/2374
  t19/71 -> concatenate/2375
  t19/72 -> concatenate/2376
  t19/73 -> concatenate/2377
  t19/74 -> concatenate/2378
  t19/75 -> concatenate/2379
  t19/76 -> concatenate/2380
  t19/77 -> concatenate/2381
  t19/78 -> concatenate/2382
  t19/79 -> concatenate/2383
  t19/80 -> concatenate/2384
  t19/81 -> concatenate/2385
  t19/82 -> concatenate/2386
  t19/83 -> concatenate/2387
  t19/84 -> concatenate/2388
  t19/85 -> concatenate/2389
  t19/86 -> concatenate/2390
  t19/87 -> concatenate/2391
  t19/88 -> concatenate/2392
  t19/89 -> concatenate/2393
  t19/90 -> concatenate/2394
  t19/91 -> concatenate/2395
  t19/92 -> concatenate/2396
  t19/93 -> concatenate/2397
  t19/94 -> concatenate/2398
  t19/95 -> concatenate/2399
  t19/96 -> concatenate/2400
  t19/97 -> concatenate/2401
  t19/98 -> concatenate/2402
  t19/99 -> concatenate/2403
  t19/100 -> concatenate/2404
  t19/101 -> concatenate/2405
  t19/102 -> concatenate/2406
  t19/103 -> concatenate/2407
  t19/104 -> concatenate/2408
  t19/105 -> concatenate/2409
  t19/106 -> concatenate/2410
  t19/107 -> concatenate/2411
  t19/108 -> concatenate/2412
  t19/109 -> concatenate/2413
  t19/110 -> concatenate/2414
  t19/111 -> concatenate/2415
  t19/112 -> concatenate/2416
  t19/113 -> concatenate/2417
  t19/114 -> concatenate/2418
  t19/115 -> concatenate/2419
  t19/116 -> concatenate/2420
  t19/117 -> concatenate/2421
  t19/118 -> concatenate/2422
  t19/119 -> concatenate/2423
  t19/120 -> concatenate/2424
  t19/121 -> concatenate/2425
  t19/122 -> concatenate/2426
  t19/123 -> concatenate/2427
  t19/124 -> concatenate/2428
  t19/125 -> concatenate/2429
  t19/126 -> concatenate/2430
  t19/127 -> concatenate/2431
  t19/128 -> concatenate/2432
  t20/1 -> concatenate/2433
  t20/2 -> concatenate/2434
  t20/3 -> concatenate/2435
  t20/4 -> concatenate/2436
  t20/5 -> concatenate/2437
  t20/6 -> concatenate/2438
  t20/7 -> concatenate/2439
  t20/8 -> concatenate/2440
  t20/9 -> concatenate/2441
  t20/10 -> concatenate/2442
  t20/11 -> concatenate/2443
  t20/12 -> concatenate/2444
  t20/13 -> concatenate/2445
  t20/14 -> concatenate/2446
  t20/15 -> concatenate/2447
  t20/16 -> concatenate/2448
  t20/17 -> concatenate/2449
  t20/18 -> concatenate/2450
  t20/19 -> concatenate/2451
  t20/20 -> concatenate/2452
  t20/21 -> concatenate/2453
  t20/22 -> concatenate/2454
  t20/23 -> concatenate/2455
  t20/24 -> concatenate/2456
  t20/25 -> concatenate/2457
  t20/26 -> concatenate/2458
  t20/27 -> concatenate/2459
  t20/28 -> concatenate/2460
  t20/29 -> concatenate/2461
  t20/30 -> concatenate/2462
  t20/31 -> concatenate/2463
  t20/32 -> concatenate/2464
  t20/33 -> concatenate/2465
  t20/34 -> concatenate/2466
  t20/35 -> concatenate/2467
  t20/36 -> concatenate/2468
  t20/37 -> concatenate/2469
  t20/38 -> concatenate/2470
  t20/39 -> concatenate/2471
  t20/40 -> concatenate/2472
  t20/41 -> concatenate/2473
  t20/42 -> concatenate/2474
  t20/43 -> concatenate/2475
  t20/44 -> concatenate/2476
  t20/45 -> concatenate/2477
  t20/46 -> concatenate/2478
  t20/47 -> concatenate/2479
  t20/48 -> concatenate/2480
  t20/49 -> concatenate/2481
  t20/50 -> concatenate/2482
  t20/51 -> concatenate/2483
  t20/52 -> concatenate/2484
  t20/53 -> concatenate/2485
  t20/54 -> concatenate/2486
  t20/55 -> concatenate/2487
  t20/56 -> concatenate/2488
  t20/57 -> concatenate/2489
  t20/58 -> concatenate/2490
  t20/59 -> concatenate/2491
  t20/60 -> concatenate/2492
  t20/61 -> concatenate/2493
  t20/62 -> concatenate/2494
  t20/63 -> concatenate/2495
  t20/64 -> concatenate/2496
  t20/65 -> concatenate/2497
  t20/66 -> concatenate/2498
  t20/67 -> concatenate/2499
  t20/68 -> concatenate/2500
  t20/69 -> concatenate/2501
  t20/70 -> concatenate/2502
  t20/71 -> concatenate/2503
  t20/72 -> concatenate/2504
  t20/73 -> concatenate/2505
  t20/74 -> concatenate/2506
  t20/75 -> concatenate/2507
  t20/76 -> concatenate/2508
  t20/77 -> concatenate/2509
  t20/78 -> concatenate/2510
  t20/79 -> concatenate/2511
  t20/80 -> concatenate/2512
  t20/81 -> concatenate/2513
  t20/82 -> concatenate/2514
  t20/83 -> concatenate/2515
  t20/84 -> concatenate/2516
  t20/85 -> concatenate/2517
  t20/86 -> concatenate/2518
  t20/87 -> concatenate/2519
  t20/88 -> concatenate/2520
  t20/89 -> concatenate/2521
  t20/90 -> concatenate/2522
  t20/91 -> concatenate/2523
  t20/92 -> concatenate/2524
  t20/93 -> concatenate/2525
  t20/94 -> concatenate/2526
  t20/95 -> concatenate/2527
  t20/96 -> concatenate/2528
  t20/97 -> concatenate/2529
  t20/98 -> concatenate/2530
  t20/99 -> concatenate/2531
  t20/100 -> concatenate/2532
  t20/101 -> concatenate/2533
  t20/102 -> concatenate/2534
  t20/103 -> concatenate/2535
  t20/104 -> concatenate/2536
  t20/105 -> concatenate/2537
  t20/106 -> concatenate/2538
  t20/107 -> concatenate/2539
  t20/108 -> concatenate/2540
  t20/109 -> concatenate/2541
  t20/110 -> concatenate/2542
  t20/111 -> concatenate/2543
  t20/112 -> concatenate/2544
  t20/113 -> concatenate/2545
  t20/114 -> concatenate/2546
  t20/115 -> concatenate/2547
  t20/116 -> concatenate/2548
  t20/117 -> concatenate/2549
  t20/118 -> concatenate/2550
  t20/119 -> concatenate/2551
  t20/120 -> concatenate/2552
  t20/121 -> concatenate/2553
  t20/122 -> concatenate/2554
  t20/123 -> concatenate/2555
  t20/124 -> concatenate/2556
  t20/125 -> concatenate/2557
  t20/126 -> concatenate/2558
  t20/127 -> concatenate/2559
  t20/128 -> concatenate/2560
  t21/1 -> concatenate/2561
  t21/2 -> concatenate/2562
  t21/3 -> concatenate/2563
  t21/4 -> concatenate/2564
  t21/5 -> concatenate/2565
  t21/6 -> concatenate/2566
  t21/7 -> concatenate/2567
  t21/8 -> concatenate/2568
  t21/9 -> concatenate/2569
  t21/10 -> concatenate/2570
  t21/11 -> concatenate/2571
  t21/12 -> concatenate/2572
  t21/13 -> concatenate/2573
  t21/14 -> concatenate/2574
  t21/15 -> concatenate/2575
  t21/16 -> concatenate/2576
  t21/17 -> concatenate/2577
  t21/18 -> concatenate/2578
  t21/19 -> concatenate/2579
  t21/20 -> concatenate/2580
  t21/21 -> concatenate/2581
  t21/22 -> concatenate/2582
  t21/23 -> concatenate/2583
  t21/24 -> concatenate/2584
  t21/25 -> concatenate/2585
  t21/26 -> concatenate/2586
  t21/27 -> concatenate/2587
  t21/28 -> concatenate/2588
  t21/29 -> concatenate/2589
  t21/30 -> concatenate/2590
  t21/31 -> concatenate/2591
  t21/32 -> concatenate/2592
  t21/33 -> concatenate/2593
  t21/34 -> concatenate/2594
  t21/35 -> concatenate/2595
  t21/36 -> concatenate/2596
  t21/37 -> concatenate/2597
  t21/38 -> concatenate/2598
  t21/39 -> concatenate/2599
  t21/40 -> concatenate/2600
  t21/41 -> concatenate/2601
  t21/42 -> concatenate/2602
  t21/43 -> concatenate/2603
  t21/44 -> concatenate/2604
  t21/45 -> concatenate/2605
  t21/46 -> concatenate/2606
  t21/47 -> concatenate/2607
  t21/48 -> concatenate/2608
  t21/49 -> concatenate/2609
  t21/50 -> concatenate/2610
  t21/51 -> concatenate/2611
  t21/52 -> concatenate/2612
  t21/53 -> concatenate/2613
  t21/54 -> concatenate/2614
  t21/55 -> concatenate/2615
  t21/56 -> concatenate/2616
  t21/57 -> concatenate/2617
  t21/58 -> concatenate/2618
  t21/59 -> concatenate/2619
  t21/60 -> concatenate/2620
  t21/61 -> concatenate/2621
  t21/62 -> concatenate/2622
  t21/63 -> concatenate/2623
  t21/64 -> concatenate/2624
  t21/65 -> concatenate/2625
  t21/66 -> concatenate/2626
  t21/67 -> concatenate/2627
  t21/68 -> concatenate/2628
  t21/69 -> concatenate/2629
  t21/70 -> concatenate/2630
  t21/71 -> concatenate/2631
  t21/72 -> concatenate/2632
  t21/73 -> concatenate/2633
  t21/74 -> concatenate/2634
  t21/75 -> concatenate/2635
  t21/76 -> concatenate/2636
  t21/77 -> concatenate/2637
  t21/78 -> concatenate/2638
  t21/79 -> concatenate/2639
  t21/80 -> concatenate/2640
  t21/81 -> concatenate/2641
  t21/82 -> concatenate/2642
  t21/83 -> concatenate/2643
  t21/84 -> concatenate/2644
  t21/85 -> concatenate/2645
  t21/86 -> concatenate/2646
  t21/87 -> concatenate/2647
  t21/88 -> concatenate/2648
  t21/89 -> concatenate/2649
  t21/90 -> concatenate/2650
  t21/91 -> concatenate/2651
  t21/92 -> concatenate/2652
  t21/93 -> concatenate/2653
  t21/94 -> concatenate/2654
  t21/95 -> concatenate/2655
  t21/96 -> concatenate/2656
  t21/97 -> concatenate/2657
  t21/98 -> concatenate/2658
  t21/99 -> concatenate/2659
  t21/100 -> concatenate/2660
  t21/101 -> concatenate/2661
  t21/102 -> concatenate/2662
  t21/103 -> concatenate/2663
  t21/104 -> concatenate/2664
  t21/105 -> concatenate/2665
  t21/106 -> concatenate/2666
  t21/107 -> concatenate/2667
  t21/108 -> concatenate/2668
  t21/109 -> concatenate/2669
  t21/110 -> concatenate/2670
  t21/111 -> concatenate/2671
  t21/112 -> concatenate/2672
  t21/113 -> concatenate/2673
  t21/114 -> concatenate/2674
  t21/115 -> concatenate/2675
  t21/116 -> concatenate/2676
  t21/117 -> concatenate/2677
  t21/118 -> concatenate/2678
  t21/119 -> concatenate/2679
  t21/120 -> concatenate/2680
  t21/121 -> concatenate/2681
  t21/122 -> concatenate/2682
  t21/123 -> concatenate/2683
  t21/124 -> concatenate/2684
  t21/125 -> concatenate/2685
  t21/126 -> concatenate/2686
  t21/127 -> concatenate/2687
  t21/128 -> concatenate/2688
  t22/1 -> concatenate/2689
  t22/2 -> concatenate/2690
  t22/3 -> concatenate/2691
  t22/4 -> concatenate/2692
  t22/5 -> concatenate/2693
  t22/6 -> concatenate/2694
  t22/7 -> concatenate/2695
  t22/8 -> concatenate/2696
  t22/9 -> concatenate/2697
  t22/10 -> concatenate/2698
  t22/11 -> concatenate/2699
  t22/12 -> concatenate/2700
  t22/13 -> concatenate/2701
  t22/14 -> concatenate/2702
  t22/15 -> concatenate/2703
  t22/16 -> concatenate/2704
  t22/17 -> concatenate/2705
  t22/18 -> concatenate/2706
  t22/19 -> concatenate/2707
  t22/20 -> concatenate/2708
  t22/21 -> concatenate/2709
  t22/22 -> concatenate/2710
  t22/23 -> concatenate/2711
  t22/24 -> concatenate/2712
  t22/25 -> concatenate/2713
  t22/26 -> concatenate/2714
  t22/27 -> concatenate/2715
  t22/28 -> concatenate/2716
  t22/29 -> concatenate/2717
  t22/30 -> concatenate/2718
  t22/31 -> concatenate/2719
  t22/32 -> concatenate/2720
  t22/33 -> concatenate/2721
  t22/34 -> concatenate/2722
  t22/35 -> concatenate/2723
  t22/36 -> concatenate/2724
  t22/37 -> concatenate/2725
  t22/38 -> concatenate/2726
  t22/39 -> concatenate/2727
  t22/40 -> concatenate/2728
  t22/41 -> concatenate/2729
  t22/42 -> concatenate/2730
  t22/43 -> concatenate/2731
  t22/44 -> concatenate/2732
  t22/45 -> concatenate/2733
  t22/46 -> concatenate/2734
  t22/47 -> concatenate/2735
  t22/48 -> concatenate/2736
  t22/49 -> concatenate/2737
  t22/50 -> concatenate/2738
  t22/51 -> concatenate/2739
  t22/52 -> concatenate/2740
  t22/53 -> concatenate/2741
  t22/54 -> concatenate/2742
  t22/55 -> concatenate/2743
  t22/56 -> concatenate/2744
  t22/57 -> concatenate/2745
  t22/58 -> concatenate/2746
  t22/59 -> concatenate/2747
  t22/60 -> concatenate/2748
  t22/61 -> concatenate/2749
  t22/62 -> concatenate/2750
  t22/63 -> concatenate/2751
  t22/64 -> concatenate/2752
  t22/65 -> concatenate/2753
  t22/66 -> concatenate/2754
  t22/67 -> concatenate/2755
  t22/68 -> concatenate/2756
  t22/69 -> concatenate/2757
  t22/70 -> concatenate/2758
  t22/71 -> concatenate/2759
  t22/72 -> concatenate/2760
  t22/73 -> concatenate/2761
  t22/74 -> concatenate/2762
  t22/75 -> concatenate/2763
  t22/76 -> concatenate/2764
  t22/77 -> concatenate/2765
  t22/78 -> concatenate/2766
  t22/79 -> concatenate/2767
  t22/80 -> concatenate/2768
  t22/81 -> concatenate/2769
  t22/82 -> concatenate/2770
  t22/83 -> concatenate/2771
  t22/84 -> concatenate/2772
  t22/85 -> concatenate/2773
  t22/86 -> concatenate/2774
  t22/87 -> concatenate/2775
  t22/88 -> concatenate/2776
  t22/89 -> concatenate/2777
  t22/90 -> concatenate/2778
  t22/91 -> concatenate/2779
  t22/92 -> concatenate/2780
  t22/93 -> concatenate/2781
  t22/94 -> concatenate/2782
  t22/95 -> concatenate/2783
  t22/96 -> concatenate/2784
  t22/97 -> concatenate/2785
  t22/98 -> concatenate/2786
  t22/99 -> concatenate/2787
  t22/100 -> concatenate/2788
  t22/101 -> concatenate/2789
  t22/102 -> concatenate/2790
  t22/103 -> concatenate/2791
  t22/104 -> concatenate/2792
  t22/105 -> concatenate/2793
  t22/106 -> concatenate/2794
  t22/107 -> concatenate/2795
  t22/108 -> concatenate/2796
  t22/109 -> concatenate/2797
  t22/110 -> concatenate/2798
  t22/111 -> concatenate/2799
  t22/112 -> concatenate/2800
  t22/113 -> concatenate/2801
  t22/114 -> concatenate/2802
  t22/115 -> concatenate/2803
  t22/116 -> concatenate/2804
  t22/117 -> concatenate/2805
  t22/118 -> concatenate/2806
  t22/119 -> concatenate/2807
  t22/120 -> concatenate/2808
  t22/121 -> concatenate/2809
  t22/122 -> concatenate/2810
  t22/123 -> concatenate/2811
  t22/124 -> concatenate/2812
  t22/125 -> concatenate/2813
  t22/126 -> concatenate/2814
  t22/127 -> concatenate/2815
  t22/128 -> concatenate/2816
  t23/1 -> concatenate/2817
  t23/2 -> concatenate/2818
  t23/3 -> concatenate/2819
  t23/4 -> concatenate/2820
  t23/5 -> concatenate/2821
  t23/6 -> concatenate/2822
  t23/7 -> concatenate/2823
  t23/8 -> concatenate/2824
  t23/9 -> concatenate/2825
  t23/10 -> concatenate/2826
  t23/11 -> concatenate/2827
  t23/12 -> concatenate/2828
  t23/13 -> concatenate/2829
  t23/14 -> concatenate/2830
  t23/15 -> concatenate/2831
  t23/16 -> concatenate/2832
  t23/17 -> concatenate/2833
  t23/18 -> concatenate/2834
  t23/19 -> concatenate/2835
  t23/20 -> concatenate/2836
  t23/21 -> concatenate/2837
  t23/22 -> concatenate/2838
  t23/23 -> concatenate/2839
  t23/24 -> concatenate/2840
  t23/25 -> concatenate/2841
  t23/26 -> concatenate/2842
  t23/27 -> concatenate/2843
  t23/28 -> concatenate/2844
  t23/29 -> concatenate/2845
  t23/30 -> concatenate/2846
  t23/31 -> concatenate/2847
  t23/32 -> concatenate/2848
  t23/33 -> concatenate/2849
  t23/34 -> concatenate/2850
  t23/35 -> concatenate/2851
  t23/36 -> concatenate/2852
  t23/37 -> concatenate/2853
  t23/38 -> concatenate/2854
  t23/39 -> concatenate/2855
  t23/40 -> concatenate/2856
  t23/41 -> concatenate/2857
  t23/42 -> concatenate/2858
  t23/43 -> concatenate/2859
  t23/44 -> concatenate/2860
  t23/45 -> concatenate/2861
  t23/46 -> concatenate/2862
  t23/47 -> concatenate/2863
  t23/48 -> concatenate/2864
  t23/49 -> concatenate/2865
  t23/50 -> concatenate/2866
  t23/51 -> concatenate/2867
  t23/52 -> concatenate/2868
  t23/53 -> concatenate/2869
  t23/54 -> concatenate/2870
  t23/55 -> concatenate/2871
  t23/56 -> concatenate/2872
  t23/57 -> concatenate/2873
  t23/58 -> concatenate/2874
  t23/59 -> concatenate/2875
  t23/60 -> concatenate/2876
  t23/61 -> concatenate/2877
  t23/62 -> concatenate/2878
  t23/63 -> concatenate/2879
  t23/64 -> concatenate/2880
  t23/65 -> concatenate/2881
  t23/66 -> concatenate/2882
  t23/67 -> concatenate/2883
  t23/68 -> concatenate/2884
  t23/69 -> concatenate/2885
  t23/70 -> concatenate/2886
  t23/71 -> concatenate/2887
  t23/72 -> concatenate/2888
  t23/73 -> concatenate/2889
  t23/74 -> concatenate/2890
  t23/75 -> concatenate/2891
  t23/76 -> concatenate/2892
  t23/77 -> concatenate/2893
  t23/78 -> concatenate/2894
  t23/79 -> concatenate/2895
  t23/80 -> concatenate/2896
  t23/81 -> concatenate/2897
  t23/82 -> concatenate/2898
  t23/83 -> concatenate/2899
  t23/84 -> concatenate/2900
  t23/85 -> concatenate/2901
  t23/86 -> concatenate/2902
  t23/87 -> concatenate/2903
  t23/88 -> concatenate/2904
  t23/89 -> concatenate/2905
  t23/90 -> concatenate/2906
  t23/91 -> concatenate/2907
  t23/92 -> concatenate/2908
  t23/93 -> concatenate/2909
  t23/94 -> concatenate/2910
  t23/95 -> concatenate/2911
  t23/96 -> concatenate/2912
  t23/97 -> concatenate/2913
  t23/98 -> concatenate/2914
  t23/99 -> concatenate/2915
  t23/100 -> concatenate/2916
  t23/101 -> concatenate/2917
  t23/102 -> concatenate/2918
  t23/103 -> concatenate/2919
  t23/104 -> concatenate/2920
  t23/105 -> concatenate/2921
  t23/106 -> concatenate/2922
  t23/107 -> concatenate/2923
  t23/108 -> concatenate/2924
  t23/109 -> concatenate/2925
  t23/110 -> concatenate/2926
  t23/111 -> concatenate/2927
  t23/112 -> concatenate/2928
  t23/113 -> concatenate/2929
  t23/114 -> concatenate/2930
  t23/115 -> concatenate/2931
  t23/116 -> concatenate/2932
  t23/117 -> concatenate/2933
  t23/118 -> concatenate/2934
  t23/119 -> concatenate/2935
  t23/120 -> concatenate/2936
  t23/121 -> concatenate/2937
  t23/122 -> concatenate/2938
  t23/123 -> concatenate/2939
  t23/124 -> concatenate/2940
  t23/125 -> concatenate/2941
  t23/126 -> concatenate/2942
  t23/127 -> concatenate/2943
  t23/128 -> concatenate/2944
  t24/1 -> concatenate/2945
  t24/2 -> concatenate/2946
  t24/3 -> concatenate/2947
  t24/4 -> concatenate/2948
  t24/5 -> concatenate/2949
  t24/6 -> concatenate/2950
  t24/7 -> concatenate/2951
  t24/8 -> concatenate/2952
  t24/9 -> concatenate/2953
  t24/10 -> concatenate/2954
  t24/11 -> concatenate/2955
  t24/12 -> concatenate/2956
  t24/13 -> concatenate/2957
  t24/14 -> concatenate/2958
  t24/15 -> concatenate/2959
  t24/16 -> concatenate/2960
  t24/17 -> concatenate/2961
  t24/18 -> concatenate/2962
  t24/19 -> concatenate/2963
  t24/20 -> concatenate/2964
  t24/21 -> concatenate/2965
  t24/22 -> concatenate/2966
  t24/23 -> concatenate/2967
  t24/24 -> concatenate/2968
  t24/25 -> concatenate/2969
  t24/26 -> concatenate/2970
  t24/27 -> concatenate/2971
  t24/28 -> concatenate/2972
  t24/29 -> concatenate/2973
  t24/30 -> concatenate/2974
  t24/31 -> concatenate/2975
  t24/32 -> concatenate/2976
  t24/33 -> concatenate/2977
  t24/34 -> concatenate/2978
  t24/35 -> concatenate/2979
  t24/36 -> concatenate/2980
  t24/37 -> concatenate/2981
  t24/38 -> concatenate/2982
  t24/39 -> concatenate/2983
  t24/40 -> concatenate/2984
  t24/41 -> concatenate/2985
  t24/42 -> concatenate/2986
  t24/43 -> concatenate/2987
  t24/44 -> concatenate/2988
  t24/45 -> concatenate/2989
  t24/46 -> concatenate/2990
  t24/47 -> concatenate/2991
  t24/48 -> concatenate/2992
  t24/49 -> concatenate/2993
  t24/50 -> concatenate/2994
  t24/51 -> concatenate/2995
  t24/52 -> concatenate/2996
  t24/53 -> concatenate/2997
  t24/54 -> concatenate/2998
  t24/55 -> concatenate/2999
  t24/56 -> concatenate/3000
  t24/57 -> concatenate/3001
  t24/58 -> concatenate/3002
  t24/59 -> concatenate/3003
  t24/60 -> concatenate/3004
  t24/61 -> concatenate/3005
  t24/62 -> concatenate/3006
  t24/63 -> concatenate/3007
  t24/64 -> concatenate/3008
  t24/65 -> concatenate/3009
  t24/66 -> concatenate/3010
  t24/67 -> concatenate/3011
  t24/68 -> concatenate/3012
  t24/69 -> concatenate/3013
  t24/70 -> concatenate/3014
  t24/71 -> concatenate/3015
  t24/72 -> concatenate/3016
  t24/73 -> concatenate/3017
  t24/74 -> concatenate/3018
  t24/75 -> concatenate/3019
  t24/76 -> concatenate/3020
  t24/77 -> concatenate/3021
  t24/78 -> concatenate/3022
  t24/79 -> concatenate/3023
  t24/80 -> concatenate/3024
  t24/81 -> concatenate/3025
  t24/82 -> concatenate/3026
  t24/83 -> concatenate/3027
  t24/84 -> concatenate/3028
  t24/85 -> concatenate/3029
  t24/86 -> concatenate/3030
  t24/87 -> concatenate/3031
  t24/88 -> concatenate/3032
  t24/89 -> concatenate/3033
  t24/90 -> concatenate/3034
  t24/91 -> concatenate/3035
  t24/92 -> concatenate/3036
  t24/93 -> concatenate/3037
  t24/94 -> concatenate/3038
  t24/95 -> concatenate/3039
  t24/96 -> concatenate/3040
  t24/97 -> concatenate/3041
  t24/98 -> concatenate/3042
  t24/99 -> concatenate/3043
  t24/100 -> concatenate/3044
  t24/101 -> concatenate/3045
  t24/102 -> concatenate/3046
  t24/103 -> concatenate/3047
  t24/104 -> concatenate/3048
  t24/105 -> concatenate/3049
  t24/106 -> concatenate/3050
  t24/107 -> concatenate/3051
  t24/108 -> concatenate/3052
  t24/109 -> concatenate/3053
  t24/110 -> concatenate/3054
  t24/111 -> concatenate/3055
  t24/112 -> concatenate/3056
  t24/113 -> concatenate/3057
  t24/114 -> concatenate/3058
  t24/115 -> concatenate/3059
  t24/116 -> concatenate/3060
  t24/117 -> concatenate/3061
  t24/118 -> concatenate/3062
  t24/119 -> concatenate/3063
  t24/120 -> concatenate/3064
  t24/121 -> concatenate/3065
  t24/122 -> concatenate/3066
  t24/123 -> concatenate/3067
  t24/124 -> concatenate/3068
  t24/125 -> concatenate/3069
  t24/126 -> concatenate/3070
  t24/127 -> concatenate/3071
  t24/128 -> concatenate/3072
  t25/1 -> concatenate/3073
  t25/2 -> concatenate/3074
  t25/3 -> concatenate/3075
  t25/4 -> concatenate/3076
  t25/5 -> concatenate/3077
  t25/6 -> concatenate/3078
  t25/7 -> concatenate/3079
  t25/8 -> concatenate/3080
  t25/9 -> concatenate/3081
  t25/10 -> concatenate/3082
  t25/11 -> concatenate/3083
  t25/12 -> concatenate/3084
  t25/13 -> concatenate/3085
  t25/14 -> concatenate/3086
  t25/15 -> concatenate/3087
  t25/16 -> concatenate/3088
  t25/17 -> concatenate/3089
  t25/18 -> concatenate/3090
  t25/19 -> concatenate/3091
  t25/20 -> concatenate/3092
  t25/21 -> concatenate/3093
  t25/22 -> concatenate/3094
  t25/23 -> concatenate/3095
  t25/24 -> concatenate/3096
  t25/25 -> concatenate/3097
  t25/26 -> concatenate/3098
  t25/27 -> concatenate/3099
  t25/28 -> concatenate/3100
  t25/29 -> concatenate/3101
  t25/30 -> concatenate/3102
  t25/31 -> concatenate/3103
  t25/32 -> concatenate/3104
  t25/33 -> concatenate/3105
  t25/34 -> concatenate/3106
  t25/35 -> concatenate/3107
  t25/36 -> concatenate/3108
  t25/37 -> concatenate/3109
  t25/38 -> concatenate/3110
  t25/39 -> concatenate/3111
  t25/40 -> concatenate/3112
  t25/41 -> concatenate/3113
  t25/42 -> concatenate/3114
  t25/43 -> concatenate/3115
  t25/44 -> concatenate/3116
  t25/45 -> concatenate/3117
  t25/46 -> concatenate/3118
  t25/47 -> concatenate/3119
  t25/48 -> concatenate/3120
  t25/49 -> concatenate/3121
  t25/50 -> concatenate/3122
  t25/51 -> concatenate/3123
  t25/52 -> concatenate/3124
  t25/53 -> concatenate/3125
  t25/54 -> concatenate/3126
  t25/55 -> concatenate/3127
  t25/56 -> concatenate/3128
  t25/57 -> concatenate/3129
  t25/58 -> concatenate/3130
  t25/59 -> concatenate/3131
  t25/60 -> concatenate/3132
  t25/61 -> concatenate/3133
  t25/62 -> concatenate/3134
  t25/63 -> concatenate/3135
  t25/64 -> concatenate/3136
  t25/65 -> concatenate/3137
  t25/66 -> concatenate/3138
  t25/67 -> concatenate/3139
  t25/68 -> concatenate/3140
  t25/69 -> concatenate/3141
  t25/70 -> concatenate/3142
  t25/71 -> concatenate/3143
  t25/72 -> concatenate/3144
  t25/73 -> concatenate/3145
  t25/74 -> concatenate/3146
  t25/75 -> concatenate/3147
  t25/76 -> concatenate/3148
  t25/77 -> concatenate/3149
  t25/78 -> concatenate/3150
  t25/79 -> concatenate/3151
  t25/80 -> concatenate/3152
  t25/81 -> concatenate/3153
  t25/82 -> concatenate/3154
  t25/83 -> concatenate/3155
  t25/84 -> concatenate/3156
  t25/85 -> concatenate/3157
  t25/86 -> concatenate/3158
  t25/87 -> concatenate/3159
  t25/88 -> concatenate/3160
  t25/89 -> concatenate/3161
  t25/90 -> concatenate/3162
  t25/91 -> concatenate/3163
  t25/92 -> concatenate/3164
  t25/93 -> concatenate/3165
  t25/94 -> concatenate/3166
  t25/95 -> concatenate/3167
  t25/96 -> concatenate/3168
  t25/97 -> concatenate/3169
  t25/98 -> concatenate/3170
  t25/99 -> concatenate/3171
  t25/100 -> concatenate/3172
  t25/101 -> concatenate/3173
  t25/102 -> concatenate/3174
  t25/103 -> concatenate/3175
  t25/104 -> concatenate/3176
  t25/105 -> concatenate/3177
  t25/106 -> concatenate/3178
  t25/107 -> concatenate/3179
  t25/108 -> concatenate/3180
  t25/109 -> concatenate/3181
  t25/110 -> concatenate/3182
  t25/111 -> concatenate/3183
  t25/112 -> concatenate/3184
  t25/113 -> concatenate/3185
  t25/114 -> concatenate/3186
  t25/115 -> concatenate/3187
  t25/116 -> concatenate/3188
  t25/117 -> concatenate/3189
  t25/118 -> concatenate/3190
  t25/119 -> concatenate/3191
  t25/120 -> concatenate/3192
  t25/121 -> concatenate/3193
  t25/122 -> concatenate/3194
  t25/123 -> concatenate/3195
  t25/124 -> concatenate/3196
  t25/125 -> concatenate/3197
  t25/126 -> concatenate/3198
  t25/127 -> concatenate/3199
  t25/128 -> concatenate/3200
  t26/1 -> concatenate/3201
  t26/2 -> concatenate/3202
  t26/3 -> concatenate/3203
  t26/4 -> concatenate/3204
  t26/5 -> concatenate/3205
  t26/6 -> concatenate/3206
  t26/7 -> concatenate/3207
  t26/8 -> concatenate/3208
  t26/9 -> concatenate/3209
  t26/10 -> concatenate/3210
  t26/11 -> concatenate/3211
  t26/12 -> concatenate/3212
  t26/13 -> concatenate/3213
  t26/14 -> concatenate/3214
  t26/15 -> concatenate/3215
  t26/16 -> concatenate/3216
  t26/17 -> concatenate/3217
  t26/18 -> concatenate/3218
  t26/19 -> concatenate/3219
  t26/20 -> concatenate/3220
  t26/21 -> concatenate/3221
  t26/22 -> concatenate/3222
  t26/23 -> concatenate/3223
  t26/24 -> concatenate/3224
  t26/25 -> concatenate/3225
  t26/26 -> concatenate/3226
  t26/27 -> concatenate/3227
  t26/28 -> concatenate/3228
  t26/29 -> concatenate/3229
  t26/30 -> concatenate/3230
  t26/31 -> concatenate/3231
  t26/32 -> concatenate/3232
  t26/33 -> concatenate/3233
  t26/34 -> concatenate/3234
  t26/35 -> concatenate/3235
  t26/36 -> concatenate/3236
  t26/37 -> concatenate/3237
  t26/38 -> concatenate/3238
  t26/39 -> concatenate/3239
  t26/40 -> concatenate/3240
  t26/41 -> concatenate/3241
  t26/42 -> concatenate/3242
  t26/43 -> concatenate/3243
  t26/44 -> concatenate/3244
  t26/45 -> concatenate/3245
  t26/46 -> concatenate/3246
  t26/47 -> concatenate/3247
  t26/48 -> concatenate/3248
  t26/49 -> concatenate/3249
  t26/50 -> concatenate/3250
  t26/51 -> concatenate/3251
  t26/52 -> concatenate/3252
  t26/53 -> concatenate/3253
  t26/54 -> concatenate/3254
  t26/55 -> concatenate/3255
  t26/56 -> concatenate/3256
  t26/57 -> concatenate/3257
  t26/58 -> concatenate/3258
  t26/59 -> concatenate/3259
  t26/60 -> concatenate/3260
  t26/61 -> concatenate/3261
  t26/62 -> concatenate/3262
  t26/63 -> concatenate/3263
  t26/64 -> concatenate/3264
  t26/65 -> concatenate/3265
  t26/66 -> concatenate/3266
  t26/67 -> concatenate/3267
  t26/68 -> concatenate/3268
  t26/69 -> concatenate/3269
  t26/70 -> concatenate/3270
  t26/71 -> concatenate/3271
  t26/72 -> concatenate/3272
  t26/73 -> concatenate/3273
  t26/74 -> concatenate/3274
  t26/75 -> concatenate/3275
  t26/76 -> concatenate/3276
  t26/77 -> concatenate/3277
  t26/78 -> concatenate/3278
  t26/79 -> concatenate/3279
  t26/80 -> concatenate/3280
  t26/81 -> concatenate/3281
  t26/82 -> concatenate/3282
  t26/83 -> concatenate/3283
  t26/84 -> concatenate/3284
  t26/85 -> concatenate/3285
  t26/86 -> concatenate/3286
  t26/87 -> concatenate/3287
  t26/88 -> concatenate/3288
  t26/89 -> concatenate/3289
  t26/90 -> concatenate/3290
  t26/91 -> concatenate/3291
  t26/92 -> concatenate/3292
  t26/93 -> concatenate/3293
  t26/94 -> concatenate/3294
  t26/95 -> concatenate/3295
  t26/96 -> concatenate/3296
  t26/97 -> concatenate/3297
  t26/98 -> concatenate/3298
  t26/99 -> concatenate/3299
  t26/100 -> concatenate/3300
  t26/101 -> concatenate/3301
  t26/102 -> concatenate/3302
  t26/103 -> concatenate/3303
  t26/104 -> concatenate/3304
  t26/105 -> concatenate/3305
  t26/106 -> concatenate/3306
  t26/107 -> concatenate/3307
  t26/108 -> concatenate/3308
  t26/109 -> concatenate/3309
  t26/110 -> concatenate/3310
  t26/111 -> concatenate/3311
  t26/112 -> concatenate/3312
  t26/113 -> concatenate/3313
  t26/114 -> concatenate/3314
  t26/115 -> concatenate/3315
  t26/116 -> concatenate/3316
  t26/117 -> concatenate/3317
  t26/118 -> concatenate/3318
  t26/119 -> concatenate/3319
  t26/120 -> concatenate/3320
  t26/121 -> concatenate/3321
  t26/122 -> concatenate/3322
  t26/123 -> concatenate/3323
  t26/124 -> concatenate/3324
  t26/125 -> concatenate/3325
  t26/126 -> concatenate/3326
  t26/127 -> concatenate/3327
  t26/128 -> concatenate/3328
  t27/1 -> concatenate/3329
  t27/2 -> concatenate/3330
  t27/3 -> concatenate/3331
  t27/4 -> concatenate/3332
  t27/5 -> concatenate/3333
  t27/6 -> concatenate/3334
  t27/7 -> concatenate/3335
  t27/8 -> concatenate/3336
  t27/9 -> concatenate/3337
  t27/10 -> concatenate/3338
  t27/11 -> concatenate/3339
  t27/12 -> concatenate/3340
  t27/13 -> concatenate/3341
  t27/14 -> concatenate/3342
  t27/15 -> concatenate/3343
  t27/16 -> concatenate/3344
  t27/17 -> concatenate/3345
  t27/18 -> concatenate/3346
  t27/19 -> concatenate/3347
  t27/20 -> concatenate/3348
  t27/21 -> concatenate/3349
  t27/22 -> concatenate/3350
  t27/23 -> concatenate/3351
  t27/24 -> concatenate/3352
  t27/25 -> concatenate/3353
  t27/26 -> concatenate/3354
  t27/27 -> concatenate/3355
  t27/28 -> concatenate/3356
  t27/29 -> concatenate/3357
  t27/30 -> concatenate/3358
  t27/31 -> concatenate/3359
  t27/32 -> concatenate/3360
  t27/33 -> concatenate/3361
  t27/34 -> concatenate/3362
  t27/35 -> concatenate/3363
  t27/36 -> concatenate/3364
  t27/37 -> concatenate/3365
  t27/38 -> concatenate/3366
  t27/39 -> concatenate/3367
  t27/40 -> concatenate/3368
  t27/41 -> concatenate/3369
  t27/42 -> concatenate/3370
  t27/43 -> concatenate/3371
  t27/44 -> concatenate/3372
  t27/45 -> concatenate/3373
  t27/46 -> concatenate/3374
  t27/47 -> concatenate/3375
  t27/48 -> concatenate/3376
  t27/49 -> concatenate/3377
  t27/50 -> concatenate/3378
  t27/51 -> concatenate/3379
  t27/52 -> concatenate/3380
  t27/53 -> concatenate/3381
  t27/54 -> concatenate/3382
  t27/55 -> concatenate/3383
  t27/56 -> concatenate/3384
  t27/57 -> concatenate/3385
  t27/58 -> concatenate/3386
  t27/59 -> concatenate/3387
  t27/60 -> concatenate/3388
  t27/61 -> concatenate/3389
  t27/62 -> concatenate/3390
  t27/63 -> concatenate/3391
  t27/64 -> concatenate/3392
  t27/65 -> concatenate/3393
  t27/66 -> concatenate/3394
  t27/67 -> concatenate/3395
  t27/68 -> concatenate/3396
  t27/69 -> concatenate/3397
  t27/70 -> concatenate/3398
  t27/71 -> concatenate/3399
  t27/72 -> concatenate/3400
  t27/73 -> concatenate/3401
  t27/74 -> concatenate/3402
  t27/75 -> concatenate/3403
  t27/76 -> concatenate/3404
  t27/77 -> concatenate/3405
  t27/78 -> concatenate/3406
  t27/79 -> concatenate/3407
  t27/80 -> concatenate/3408
  t27/81 -> concatenate/3409
  t27/82 -> concatenate/3410
  t27/83 -> concatenate/3411
  t27/84 -> concatenate/3412
  t27/85 -> concatenate/3413
  t27/86 -> concatenate/3414
  t27/87 -> concatenate/3415
  t27/88 -> concatenate/3416
  t27/89 -> concatenate/3417
  t27/90 -> concatenate/3418
  t27/91 -> concatenate/3419
  t27/92 -> concatenate/3420
  t27/93 -> concatenate/3421
  t27/94 -> concatenate/3422
  t27/95 -> concatenate/3423
  t27/96 -> concatenate/3424
  t27/97 -> concatenate/3425
  t27/98 -> concatenate/3426
  t27/99 -> concatenate/3427
  t27/100 -> concatenate/3428
  t27/101 -> concatenate/3429
  t27/102 -> concatenate/3430
  t27/103 -> concatenate/3431
  t27/104 -> concatenate/3432
  t27/105 -> concatenate/3433
  t27/106 -> concatenate/3434
  t27/107 -> concatenate/3435
  t27/108 -> concatenate/3436
  t27/109 -> concatenate/3437
  t27/110 -> concatenate/3438
  t27/111 -> concatenate/3439
  t27/112 -> concatenate/3440
  t27/113 -> concatenate/3441
  t27/114 -> concatenate/3442
  t27/115 -> concatenate/3443
  t27/116 -> concatenate/3444
  t27/117 -> concatenate/3445
  t27/118 -> concatenate/3446
  t27/119 -> concatenate/3447
  t27/120 -> concatenate/3448
  t27/121 -> concatenate/3449
  t27/122 -> concatenate/3450
  t27/123 -> concatenate/3451
  t27/124 -> concatenate/3452
  t27/125 -> concatenate/3453
  t27/126 -> concatenate/3454
  t27/127 -> concatenate/3455
  t27/128 -> concatenate/3456
  t28/1 -> concatenate/3457
  t28/2 -> concatenate/3458
  t28/3 -> concatenate/3459
  t28/4 -> concatenate/3460
  t28/5 -> concatenate/3461
  t28/6 -> concatenate/3462
  t28/7 -> concatenate/3463
  t28/8 -> concatenate/3464
  t28/9 -> concatenate/3465
  t28/10 -> concatenate/3466
  t28/11 -> concatenate/3467
  t28/12 -> concatenate/3468
  t28/13 -> concatenate/3469
  t28/14 -> concatenate/3470
  t28/15 -> concatenate/3471
  t28/16 -> concatenate/3472
  t28/17 -> concatenate/3473
  t28/18 -> concatenate/3474
  t28/19 -> concatenate/3475
  t28/20 -> concatenate/3476
  t28/21 -> concatenate/3477
  t28/22 -> concatenate/3478
  t28/23 -> concatenate/3479
  t28/24 -> concatenate/3480
  t28/25 -> concatenate/3481
  t28/26 -> concatenate/3482
  t28/27 -> concatenate/3483
  t28/28 -> concatenate/3484
  t28/29 -> concatenate/3485
  t28/30 -> concatenate/3486
  t28/31 -> concatenate/3487
  t28/32 -> concatenate/3488
  t28/33 -> concatenate/3489
  t28/34 -> concatenate/3490
  t28/35 -> concatenate/3491
  t28/36 -> concatenate/3492
  t28/37 -> concatenate/3493
  t28/38 -> concatenate/3494
  t28/39 -> concatenate/3495
  t28/40 -> concatenate/3496
  t28/41 -> concatenate/3497
  t28/42 -> concatenate/3498
  t28/43 -> concatenate/3499
  t28/44 -> concatenate/3500
  t28/45 -> concatenate/3501
  t28/46 -> concatenate/3502
  t28/47 -> concatenate/3503
  t28/48 -> concatenate/3504
  t28/49 -> concatenate/3505
  t28/50 -> concatenate/3506
  t28/51 -> concatenate/3507
  t28/52 -> concatenate/3508
  t28/53 -> concatenate/3509
  t28/54 -> concatenate/3510
  t28/55 -> concatenate/3511
  t28/56 -> concatenate/3512
  t28/57 -> concatenate/3513
  t28/58 -> concatenate/3514
  t28/59 -> concatenate/3515
  t28/60 -> concatenate/3516
  t28/61 -> concatenate/3517
  t28/62 -> concatenate/3518
  t28/63 -> concatenate/3519
  t28/64 -> concatenate/3520
  t28/65 -> concatenate/3521
  t28/66 -> concatenate/3522
  t28/67 -> concatenate/3523
  t28/68 -> concatenate/3524
  t28/69 -> concatenate/3525
  t28/70 -> concatenate/3526
  t28/71 -> concatenate/3527
  t28/72 -> concatenate/3528
  t28/73 -> concatenate/3529
  t28/74 -> concatenate/3530
  t28/75 -> concatenate/3531
  t28/76 -> concatenate/3532
  t28/77 -> concatenate/3533
  t28/78 -> concatenate/3534
  t28/79 -> concatenate/3535
  t28/80 -> concatenate/3536
  t28/81 -> concatenate/3537
  t28/82 -> concatenate/3538
  t28/83 -> concatenate/3539
  t28/84 -> concatenate/3540
  t28/85 -> concatenate/3541
  t28/86 -> concatenate/3542
  t28/87 -> concatenate/3543
  t28/88 -> concatenate/3544
  t28/89 -> concatenate/3545
  t28/90 -> concatenate/3546
  t28/91 -> concatenate/3547
  t28/92 -> concatenate/3548
  t28/93 -> concatenate/3549
  t28/94 -> concatenate/3550
  t28/95 -> concatenate/3551
  t28/96 -> concatenate/3552
  t28/97 -> concatenate/3553
  t28/98 -> concatenate/3554
  t28/99 -> concatenate/3555
  t28/100 -> concatenate/3556
  t28/101 -> concatenate/3557
  t28/102 -> concatenate/3558
  t28/103 -> concatenate/3559
  t28/104 -> concatenate/3560
  t28/105 -> concatenate/3561
  t28/106 -> concatenate/3562
  t28/107 -> concatenate/3563
  t28/108 -> concatenate/3564
  t28/109 -> concatenate/3565
  t28/110 -> concatenate/3566
  t28/111 -> concatenate/3567
  t28/112 -> concatenate/3568
  t28/113 -> concatenate/3569
  t28/114 -> concatenate/3570
  t28/115 -> concatenate/3571
  t28/116 -> concatenate/3572
  t28/117 -> concatenate/3573
  t28/118 -> concatenate/3574
  t28/119 -> concatenate/3575
  t28/120 -> concatenate/3576
  t28/121 -> concatenate/3577
  t28/122 -> concatenate/3578
  t28/123 -> concatenate/3579
  t28/124 -> concatenate/3580
  t28/125 -> concatenate/3581
  t28/126 -> concatenate/3582
  t28/127 -> concatenate/3583
  t28/128 -> concatenate/3584
  t29/1 -> concatenate/3585
  t29/2 -> concatenate/3586
  t29/3 -> concatenate/3587
  t29/4 -> concatenate/3588
  t29/5 -> concatenate/3589
  t29/6 -> concatenate/3590
  t29/7 -> concatenate/3591
  t29/8 -> concatenate/3592
  t29/9 -> concatenate/3593
  t29/10 -> concatenate/3594
  t29/11 -> concatenate/3595
  t29/12 -> concatenate/3596
  t29/13 -> concatenate/3597
  t29/14 -> concatenate/3598
  t29/15 -> concatenate/3599
  t29/16 -> concatenate/3600
  t29/17 -> concatenate/3601
  t29/18 -> concatenate/3602
  t29/19 -> concatenate/3603
  t29/20 -> concatenate/3604
  t29/21 -> concatenate/3605
  t29/22 -> concatenate/3606
  t29/23 -> concatenate/3607
  t29/24 -> concatenate/3608
  t29/25 -> concatenate/3609
  t29/26 -> concatenate/3610
  t29/27 -> concatenate/3611
  t29/28 -> concatenate/3612
  t29/29 -> concatenate/3613
  t29/30 -> concatenate/3614
  t29/31 -> concatenate/3615
  t29/32 -> concatenate/3616
  t29/33 -> concatenate/3617
  t29/34 -> concatenate/3618
  t29/35 -> concatenate/3619
  t29/36 -> concatenate/3620
  t29/37 -> concatenate/3621
  t29/38 -> concatenate/3622
  t29/39 -> concatenate/3623
  t29/40 -> concatenate/3624
  t29/41 -> concatenate/3625
  t29/42 -> concatenate/3626
  t29/43 -> concatenate/3627
  t29/44 -> concatenate/3628
  t29/45 -> concatenate/3629
  t29/46 -> concatenate/3630
  t29/47 -> concatenate/3631
  t29/48 -> concatenate/3632
  t29/49 -> concatenate/3633
  t29/50 -> concatenate/3634
  t29/51 -> concatenate/3635
  t29/52 -> concatenate/3636
  t29/53 -> concatenate/3637
  t29/54 -> concatenate/3638
  t29/55 -> concatenate/3639
  t29/56 -> concatenate/3640
  t29/57 -> concatenate/3641
  t29/58 -> concatenate/3642
  t29/59 -> concatenate/3643
  t29/60 -> concatenate/3644
  t29/61 -> concatenate/3645
  t29/62 -> concatenate/3646
  t29/63 -> concatenate/3647
  t29/64 -> concatenate/3648
  t29/65 -> concatenate/3649
  t29/66 -> concatenate/3650
  t29/67 -> concatenate/3651
  t29/68 -> concatenate/3652
  t29/69 -> concatenate/3653
  t29/70 -> concatenate/3654
  t29/71 -> concatenate/3655
  t29/72 -> concatenate/3656
  t29/73 -> concatenate/3657
  t29/74 -> concatenate/3658
  t29/75 -> concatenate/3659
  t29/76 -> concatenate/3660
  t29/77 -> concatenate/3661
  t29/78 -> concatenate/3662
  t29/79 -> concatenate/3663
  t29/80 -> concatenate/3664
  t29/81 -> concatenate/3665
  t29/82 -> concatenate/3666
  t29/83 -> concatenate/3667
  t29/84 -> concatenate/3668
  t29/85 -> concatenate/3669
  t29/86 -> concatenate/3670
  t29/87 -> concatenate/3671
  t29/88 -> concatenate/3672
  t29/89 -> concatenate/3673
  t29/90 -> concatenate/3674
  t29/91 -> concatenate/3675
  t29/92 -> concatenate/3676
  t29/93 -> concatenate/3677
  t29/94 -> concatenate/3678
  t29/95 -> concatenate/3679
  t29/96 -> concatenate/3680
  t29/97 -> concatenate/3681
  t29/98 -> concatenate/3682
  t29/99 -> concatenate/3683
  t29/100 -> concatenate/3684
  t29/101 -> concatenate/3685
  t29/102 -> concatenate/3686
  t29/103 -> concatenate/3687
  t29/104 -> concatenate/3688
  t29/105 -> concatenate/3689
  t29/106 -> concatenate/3690
  t29/107 -> concatenate/3691
  t29/108 -> concatenate/3692
  t29/109 -> concatenate/3693
  t29/110 -> concatenate/3694
  t29/111 -> concatenate/3695
  t29/112 -> concatenate/3696
  t29/113 -> concatenate/3697
  t29/114 -> concatenate/3698
  t29/115 -> concatenate/3699
  t29/116 -> concatenate/3700
  t29/117 -> concatenate/3701
  t29/118 -> concatenate/3702
  t29/119 -> concatenate/3703
  t29/120 -> concatenate/3704
  t29/121 -> concatenate/3705
  t29/122 -> concatenate/3706
  t29/123 -> concatenate/3707
  t29/124 -> concatenate/3708
  t29/125 -> concatenate/3709
  t29/126 -> concatenate/3710
  t29/127 -> concatenate/3711
  t29/128 -> concatenate/3712
  t30/1 -> concatenate/3713
  t30/2 -> concatenate/3714
  t30/3 -> concatenate/3715
  t30/4 -> concatenate/3716
  t30/5 -> concatenate/3717
  t30/6 -> concatenate/3718
  t30/7 -> concatenate/3719
  t30/8 -> concatenate/3720
  t30/9 -> concatenate/3721
  t30/10 -> concatenate/3722
  t30/11 -> concatenate/3723
  t30/12 -> concatenate/3724
  t30/13 -> concatenate/3725
  t30/14 -> concatenate/3726
  t30/15 -> concatenate/3727
  t30/16 -> concatenate/3728
  t30/17 -> concatenate/3729
  t30/18 -> concatenate/3730
  t30/19 -> concatenate/3731
  t30/20 -> concatenate/3732
  t30/21 -> concatenate/3733
  t30/22 -> concatenate/3734
  t30/23 -> concatenate/3735
  t30/24 -> concatenate/3736
  t30/25 -> concatenate/3737
  t30/26 -> concatenate/3738
  t30/27 -> concatenate/3739
  t30/28 -> concatenate/3740
  t30/29 -> concatenate/3741
  t30/30 -> concatenate/3742
  t30/31 -> concatenate/3743
  t30/32 -> concatenate/3744
  t30/33 -> concatenate/3745
  t30/34 -> concatenate/3746
  t30/35 -> concatenate/3747
  t30/36 -> concatenate/3748
  t30/37 -> concatenate/3749
  t30/38 -> concatenate/3750
  t30/39 -> concatenate/3751
  t30/40 -> concatenate/3752
  t30/41 -> concatenate/3753
  t30/42 -> concatenate/3754
  t30/43 -> concatenate/3755
  t30/44 -> concatenate/3756
  t30/45 -> concatenate/3757
  t30/46 -> concatenate/3758
  t30/47 -> concatenate/3759
  t30/48 -> concatenate/3760
  t30/49 -> concatenate/3761
  t30/50 -> concatenate/3762
  t30/51 -> concatenate/3763
  t30/52 -> concatenate/3764
  t30/53 -> concatenate/3765
  t30/54 -> concatenate/3766
  t30/55 -> concatenate/3767
  t30/56 -> concatenate/3768
  t30/57 -> concatenate/3769
  t30/58 -> concatenate/3770
  t30/59 -> concatenate/3771
  t30/60 -> concatenate/3772
  t30/61 -> concatenate/3773
  t30/62 -> concatenate/3774
  t30/63 -> concatenate/3775
  t30/64 -> concatenate/3776
  t30/65 -> concatenate/3777
  t30/66 -> concatenate/3778
  t30/67 -> concatenate/3779
  t30/68 -> concatenate/3780
  t30/69 -> concatenate/3781
  t30/70 -> concatenate/3782
  t30/71 -> concatenate/3783
  t30/72 -> concatenate/3784
  t30/73 -> concatenate/3785
  t30/74 -> concatenate/3786
  t30/75 -> concatenate/3787
  t30/76 -> concatenate/3788
  t30/77 -> concatenate/3789
  t30/78 -> concatenate/3790
  t30/79 -> concatenate/3791
  t30/80 -> concatenate/3792
  t30/81 -> concatenate/3793
  t30/82 -> concatenate/3794
  t30/83 -> concatenate/3795
  t30/84 -> concatenate/3796
  t30/85 -> concatenate/3797
  t30/86 -> concatenate/3798
  t30/87 -> concatenate/3799
  t30/88 -> concatenate/3800
  t30/89 -> concatenate/3801
  t30/90 -> concatenate/3802
  t30/91 -> concatenate/3803
  t30/92 -> concatenate/3804
  t30/93 -> concatenate/3805
  t30/94 -> concatenate/3806
  t30/95 -> concatenate/3807
  t30/96 -> concatenate/3808
  t30/97 -> concatenate/3809
  t30/98 -> concatenate/3810
  t30/99 -> concatenate/3811
  t30/100 -> concatenate/3812
  t30/101 -> concatenate/3813
  t30/102 -> concatenate/3814
  t30/103 -> concatenate/3815
  t30/104 -> concatenate/3816
  t30/105 -> concatenate/3817
  t30/106 -> concatenate/3818
  t30/107 -> concatenate/3819
  t30/108 -> concatenate/3820
  t30/109 -> concatenate/3821
  t30/110 -> concatenate/3822
  t30/111 -> concatenate/3823
  t30/112 -> concatenate/3824
  t30/113 -> concatenate/3825
  t30/114 -> concatenate/3826
  t30/115 -> concatenate/3827
  t30/116 -> concatenate/3828
  t30/117 -> concatenate/3829
  t30/118 -> concatenate/3830
  t30/119 -> concatenate/3831
  t30/120 -> concatenate/3832
  t30/121 -> concatenate/3833
  t30/122 -> concatenate/3834
  t30/123 -> concatenate/3835
  t30/124 -> concatenate/3836
  t30/125 -> concatenate/3837
  t30/126 -> concatenate/3838
  t30/127 -> concatenate/3839
  t30/128 -> concatenate/3840
  t31/1 -> concatenate/3841
  t31/2 -> concatenate/3842
  t31/3 -> concatenate/3843
  t31/4 -> concatenate/3844
  t31/5 -> concatenate/3845
  t31/6 -> concatenate/3846
  t31/7 -> concatenate/3847
  t31/8 -> concatenate/3848
  t31/9 -> concatenate/3849
  t31/10 -> concatenate/3850
  t31/11 -> concatenate/3851
  t31/12 -> concatenate/3852
  t31/13 -> concatenate/3853
  t31/14 -> concatenate/3854
  t31/15 -> concatenate/3855
  t31/16 -> concatenate/3856
  t31/17 -> concatenate/3857
  t31/18 -> concatenate/3858
  t31/19 -> concatenate/3859
  t31/20 -> concatenate/3860
  t31/21 -> concatenate/3861
  t31/22 -> concatenate/3862
  t31/23 -> concatenate/3863
  t31/24 -> concatenate/3864
  t31/25 -> concatenate/3865
  t31/26 -> concatenate/3866
  t31/27 -> concatenate/3867
  t31/28 -> concatenate/3868
  t31/29 -> concatenate/3869
  t31/30 -> concatenate/3870
  t31/31 -> concatenate/3871
  t31/32 -> concatenate/3872
  t31/33 -> concatenate/3873
  t31/34 -> concatenate/3874
  t31/35 -> concatenate/3875
  t31/36 -> concatenate/3876
  t31/37 -> concatenate/3877
  t31/38 -> concatenate/3878
  t31/39 -> concatenate/3879
  t31/40 -> concatenate/3880
  t31/41 -> concatenate/3881
  t31/42 -> concatenate/3882
  t31/43 -> concatenate/3883
  t31/44 -> concatenate/3884
  t31/45 -> concatenate/3885
  t31/46 -> concatenate/3886
  t31/47 -> concatenate/3887
  t31/48 -> concatenate/3888
  t31/49 -> concatenate/3889
  t31/50 -> concatenate/3890
  t31/51 -> concatenate/3891
  t31/52 -> concatenate/3892
  t31/53 -> concatenate/3893
  t31/54 -> concatenate/3894
  t31/55 -> concatenate/3895
  t31/56 -> concatenate/3896
  t31/57 -> concatenate/3897
  t31/58 -> concatenate/3898
  t31/59 -> concatenate/3899
  t31/60 -> concatenate/3900
  t31/61 -> concatenate/3901
  t31/62 -> concatenate/3902
  t31/63 -> concatenate/3903
  t31/64 -> concatenate/3904
  t31/65 -> concatenate/3905
  t31/66 -> concatenate/3906
  t31/67 -> concatenate/3907
  t31/68 -> concatenate/3908
  t31/69 -> concatenate/3909
  t31/70 -> concatenate/3910
  t31/71 -> concatenate/3911
  t31/72 -> concatenate/3912
  t31/73 -> concatenate/3913
  t31/74 -> concatenate/3914
  t31/75 -> concatenate/3915
  t31/76 -> concatenate/3916
  t31/77 -> concatenate/3917
  t31/78 -> concatenate/3918
  t31/79 -> concatenate/3919
  t31/80 -> concatenate/3920
  t31/81 -> concatenate/3921
  t31/82 -> concatenate/3922
  t31/83 -> concatenate/3923
  t31/84 -> concatenate/3924
  t31/85 -> concatenate/3925
  t31/86 -> concatenate/3926
  t31/87 -> concatenate/3927
  t31/88 -> concatenate/3928
  t31/89 -> concatenate/3929
  t31/90 -> concatenate/3930
  t31/91 -> concatenate/3931
  t31/92 -> concatenate/3932
  t31/93 -> concatenate/3933
  t31/94 -> concatenate/3934
  t31/95 -> concatenate/3935
  t31/96 -> concatenate/3936
  t31/97 -> concatenate/3937
  t31/98 -> concatenate/3938
  t31/99 -> concatenate/3939
  t31/100 -> concatenate/3940
  t31/101 -> concatenate/3941
  t31/102 -> concatenate/3942
  t31/103 -> concatenate/3943
  t31/104 -> concatenate/3944
  t31/105 -> concatenate/3945
  t31/106 -> concatenate/3946
  t31/107 -> concatenate/3947
  t31/108 -> concatenate/3948
  t31/109 -> concatenate/3949
  t31/110 -> concatenate/3950
  t31/111 -> concatenate/3951
  t31/112 -> concatenate/3952
  t31/113 -> concatenate/3953
  t31/114 -> concatenate/3954
  t31/115 -> concatenate/3955
  t31/116 -> concatenate/3956
  t31/117 -> concatenate/3957
  t31/118 -> concatenate/3958
  t31/119 -> concatenate/3959
  t31/120 -> concatenate/3960
  t31/121 -> concatenate/3961
  t31/122 -> concatenate/3962
  t31/123 -> concatenate/3963
  t31/124 -> concatenate/3964
  t31/125 -> concatenate/3965
  t31/126 -> concatenate/3966
  t31/127 -> concatenate/3967
  t31/128 -> concatenate/3968
  t32/1 -> concatenate/3969
  t32/2 -> concatenate/3970
  t32/3 -> concatenate/3971
  t32/4 -> concatenate/3972
  t32/5 -> concatenate/3973
  t32/6 -> concatenate/3974
  t32/7 -> concatenate/3975
  t32/8 -> concatenate/3976
  t32/9 -> concatenate/3977
  t32/10 -> concatenate/3978
  t32/11 -> concatenate/3979
  t32/12 -> concatenate/3980
  t32/13 -> concatenate/3981
  t32/14 -> concatenate/3982
  t32/15 -> concatenate/3983
  t32/16 -> concatenate/3984
  t32/17 -> concatenate/3985
  t32/18 -> concatenate/3986
  t32/19 -> concatenate/3987
  t32/20 -> concatenate/3988
  t32/21 -> concatenate/3989
  t32/22 -> concatenate/3990
  t32/23 -> concatenate/3991
  t32/24 -> concatenate/3992
  t32/25 -> concatenate/3993
  t32/26 -> concatenate/3994
  t32/27 -> concatenate/3995
  t32/28 -> concatenate/3996
  t32/29 -> concatenate/3997
  t32/30 -> concatenate/3998
  t32/31 -> concatenate/3999
  t32/32 -> concatenate/4000
  t32/33 -> concatenate/4001
  t32/34 -> concatenate/4002
  t32/35 -> concatenate/4003
  t32/36 -> concatenate/4004
  t32/37 -> concatenate/4005
  t32/38 -> concatenate/4006
  t32/39 -> concatenate/4007
  t32/40 -> concatenate/4008
  t32/41 -> concatenate/4009
  t32/42 -> concatenate/4010
  t32/43 -> concatenate/4011
  t32/44 -> concatenate/4012
  t32/45 -> concatenate/4013
  t32/46 -> concatenate/4014
  t32/47 -> concatenate/4015
  t32/48 -> concatenate/4016
  t32/49 -> concatenate/4017
  t32/50 -> concatenate/4018
  t32/51 -> concatenate/4019
  t32/52 -> concatenate/4020
  t32/53 -> concatenate/4021
  t32/54 -> concatenate/4022
  t32/55 -> concatenate/4023
  t32/56 -> concatenate/4024
  t32/57 -> concatenate/4025
  t32/58 -> concatenate/4026
  t32/59 -> concatenate/4027
  t32/60 -> concatenate/4028
  t32/61 -> concatenate/4029
  t32/62 -> concatenate/4030
  t32/63 -> concatenate/4031
  t32/64 -> concatenate/4032
  t32/65 -> concatenate/4033
  t32/66 -> concatenate/4034
  t32/67 -> concatenate/4035
  t32/68 -> concatenate/4036
  t32/69 -> concatenate/4037
  t32/70 -> concatenate/4038
  t32/71 -> concatenate/4039
  t32/72 -> concatenate/4040
  t32/73 -> concatenate/4041
  t32/74 -> concatenate/4042
  t32/75 -> concatenate/4043
  t32/76 -> concatenate/4044
  t32/77 -> concatenate/4045
  t32/78 -> concatenate/4046
  t32/79 -> concatenate/4047
  t32/80 -> concatenate/4048
  t32/81 -> concatenate/4049
  t32/82 -> concatenate/4050
  t32/83 -> concatenate/4051
  t32/84 -> concatenate/4052
  t32/85 -> concatenate/4053
  t32/86 -> concatenate/4054
  t32/87 -> concatenate/4055
  t32/88 -> concatenate/4056
  t32/89 -> concatenate/4057
  t32/90 -> concatenate/4058
  t32/91 -> concatenate/4059
  t32/92 -> concatenate/4060
  t32/93 -> concatenate/4061
  t32/94 -> concatenate/4062
  t32/95 -> concatenate/4063
  t32/96 -> concatenate/4064
  t32/97 -> concatenate/4065
  t32/98 -> concatenate/4066
  t32/99 -> concatenate/4067
  t32/100 -> concatenate/4068
  t32/101 -> concatenate/4069
  t32/102 -> concatenate/4070
  t32/103 -> concatenate/4071
  t32/104 -> concatenate/4072
  t32/105 -> concatenate/4073
  t32/106 -> concatenate/4074
  t32/107 -> concatenate/4075
  t32/108 -> concatenate/4076
  t32/109 -> concatenate/4077
  t32/110 -> concatenate/4078
  t32/111 -> concatenate/4079
  t32/112 -> concatenate/4080
  t32/113 -> concatenate/4081
  t32/114 -> concatenate/4082
  t32/115 -> concatenate/4083
  t32/116 -> concatenate/4084
  t32/117 -> concatenate/4085
  t32/118 -> concatenate/4086
  t32/119 -> concatenate/4087
  t32/120 -> concatenate/4088
  t32/121 -> concatenate/4089
  t32/122 -> concatenate/4090
  t32/123 -> concatenate/4091
  t32/124 -> concatenate/4092
  t32/125 -> concatenate/4093
  t32/126 -> concatenate/4094
  t32/127 -> concatenate/4095
  t32/128 -> concatenate/4096
  t33/1 -> concatenate/4097
  t33/2 -> concatenate/4098
  t33/3 -> concatenate/4099
  t33/4 -> concatenate/4100
  t33/5 -> concatenate/4101
  t33/6 -> concatenate/4102
  t33/7 -> concatenate/4103
  t33/8 -> concatenate/4104
  t33/9 -> concatenate/4105
  t33/10 -> concatenate/4106
  t33/11 -> concatenate/4107
  t33/12 -> concatenate/4108
  t33/13 -> concatenate/4109
  t33/14 -> concatenate/4110
  t33/15 -> concatenate/4111
  t33/16 -> concatenate/4112
  t33/17 -> concatenate/4113
  t33/18 -> concatenate/4114
  t33/19 -> concatenate/4115
  t33/20 -> concatenate/4116
  t33/21 -> concatenate/4117
  t33/22 -> concatenate/4118
  t33/23 -> concatenate/4119
  t33/24 -> concatenate/4120
  t33/25 -> concatenate/4121
  t33/26 -> concatenate/4122
  t33/27 -> concatenate/4123
  t33/28 -> concatenate/4124
  t33/29 -> concatenate/4125
  t33/30 -> concatenate/4126
  t33/31 -> concatenate/4127
  t33/32 -> concatenate/4128
  t33/33 -> concatenate/4129
  t33/34 -> concatenate/4130
  t33/35 -> concatenate/4131
  t33/36 -> concatenate/4132
  t33/37 -> concatenate/4133
  t33/38 -> concatenate/4134
  t33/39 -> concatenate/4135
  t33/40 -> concatenate/4136
  t33/41 -> concatenate/4137
  t33/42 -> concatenate/4138
  t33/43 -> concatenate/4139
  t33/44 -> concatenate/4140
  t33/45 -> concatenate/4141
  t33/46 -> concatenate/4142
  t33/47 -> concatenate/4143
  t33/48 -> concatenate/4144
  t33/49 -> concatenate/4145
  t33/50 -> concatenate/4146
  t33/51 -> concatenate/4147
  t33/52 -> concatenate/4148
  t33/53 -> concatenate/4149
  t33/54 -> concatenate/4150
  t33/55 -> concatenate/4151
  t33/56 -> concatenate/4152
  t33/57 -> concatenate/4153
  t33/58 -> concatenate/4154
  t33/59 -> concatenate/4155
  t33/60 -> concatenate/4156
  t33/61 -> concatenate/4157
  t33/62 -> concatenate/4158
  t33/63 -> concatenate/4159
  t33/64 -> concatenate/4160
  t33/65 -> concatenate/4161
  t33/66 -> concatenate/4162
  t33/67 -> concatenate/4163
  t33/68 -> concatenate/4164
  t33/69 -> concatenate/4165
  t33/70 -> concatenate/4166
  t33/71 -> concatenate/4167
  t33/72 -> concatenate/4168
  t33/73 -> concatenate/4169
  t33/74 -> concatenate/4170
  t33/75 -> concatenate/4171
  t33/76 -> concatenate/4172
  t33/77 -> concatenate/4173
  t33/78 -> concatenate/4174
  t33/79 -> concatenate/4175
  t33/80 -> concatenate/4176
  t33/81 -> concatenate/4177
  t33/82 -> concatenate/4178
  t33/83 -> concatenate/4179
  t33/84 -> concatenate/4180
  t33/85 -> concatenate/4181
  t33/86 -> concatenate/4182
  t33/87 -> concatenate/4183
  t33/88 -> concatenate/4184
  t33/89 -> concatenate/4185
  t33/90 -> concatenate/4186
  t33/91 -> concatenate/4187
  t33/92 -> concatenate/4188
  t33/93 -> concatenate/4189
  t33/94 -> concatenate/4190
  t33/95 -> concatenate/4191
  t33/96 -> concatenate/4192
  t33/97 -> concatenate/4193
  t33/98 -> concatenate/4194
  t33/99 -> concatenate/4195
  t33/100 -> concatenate/4196
  t33/101 -> concatenate/4197
  t33/102 -> concatenate/4198
  t33/103 -> concatenate/4199
  t33/104 -> concatenate/4200
  t33/105 -> concatenate/4201
  t33/106 -> concatenate/4202
  t33/107 -> concatenate/4203
  t33/108 -> concatenate/4204
  t33/109 -> concatenate/4205
  t33/110 -> concatenate/4206
  t33/111 -> concatenate/4207
  t33/112 -> concatenate/4208
  t33/113 -> concatenate/4209
  t33/114 -> concatenate/4210
  t33/115 -> concatenate/4211
  t33/116 -> concatenate/4212
  t33/117 -> concatenate/4213
  t33/118 -> concatenate/4214
  t33/119 -> concatenate/4215
  t33/120 -> concatenate/4216
  t33/121 -> concatenate/4217
  t33/122 -> concatenate/4218
  t33/123 -> concatenate/4219
  t33/124 -> concatenate/4220
  t33/125 -> concatenate/4221
  t33/126 -> concatenate/4222
  t33/127 -> concatenate/4223
  t33/128 -> concatenate/4224
  t34/1 -> concatenate/4225
  t34/2 -> concatenate/4226
  t34/3 -> concatenate/4227
  t34/4 -> concatenate/4228
  t34/5 -> concatenate/4229
  t34/6 -> concatenate/4230
  t34/7 -> concatenate/4231
  t34/8 -> concatenate/4232
  t34/9 -> concatenate/4233
  t34/10 -> concatenate/4234
  t34/11 -> concatenate/4235
  t34/12 -> concatenate/4236
  t34/13 -> concatenate/4237
  t34/14 -> concatenate/4238
  t34/15 -> concatenate/4239
  t34/16 -> concatenate/4240
  t34/17 -> concatenate/4241
  t34/18 -> concatenate/4242
  t34/19 -> concatenate/4243
  t34/20 -> concatenate/4244
  t34/21 -> concatenate/4245
  t34/22 -> concatenate/4246
  t34/23 -> concatenate/4247
  t34/24 -> concatenate/4248
  t34/25 -> concatenate/4249
  t34/26 -> concatenate/4250
  t34/27 -> concatenate/4251
  t34/28 -> concatenate/4252
  t34/29 -> concatenate/4253
  t34/30 -> concatenate/4254
  t34/31 -> concatenate/4255
  t34/32 -> concatenate/4256
  t34/33 -> concatenate/4257
  t34/34 -> concatenate/4258
  t34/35 -> concatenate/4259
  t34/36 -> concatenate/4260
  t34/37 -> concatenate/4261
  t34/38 -> concatenate/4262
  t34/39 -> concatenate/4263
  t34/40 -> concatenate/4264
  t34/41 -> concatenate/4265
  t34/42 -> concatenate/4266
  t34/43 -> concatenate/4267
  t34/44 -> concatenate/4268
  t34/45 -> concatenate/4269
  t34/46 -> concatenate/4270
  t34/47 -> concatenate/4271
  t34/48 -> concatenate/4272
  t34/49 -> concatenate/4273
  t34/50 -> concatenate/4274
  t34/51 -> concatenate/4275
  t34/52 -> concatenate/4276
  t34/53 -> concatenate/4277
  t34/54 -> concatenate/4278
  t34/55 -> concatenate/4279
  t34/56 -> concatenate/4280
  t34/57 -> concatenate/4281
  t34/58 -> concatenate/4282
  t34/59 -> concatenate/4283
  t34/60 -> concatenate/4284
  t34/61 -> concatenate/4285
  t34/62 -> concatenate/4286
  t34/63 -> concatenate/4287
  t34/64 -> concatenate/4288
  t34/65 -> concatenate/4289
  t34/66 -> concatenate/4290
  t34/67 -> concatenate/4291
  t34/68 -> concatenate/4292
  t34/69 -> concatenate/4293
  t34/70 -> concatenate/4294
  t34/71 -> concatenate/4295
  t34/72 -> concatenate/4296
  t34/73 -> concatenate/4297
  t34/74 -> concatenate/4298
  t34/75 -> concatenate/4299
  t34/76 -> concatenate/4300
  t34/77 -> concatenate/4301
  t34/78 -> concatenate/4302
  t34/79 -> concatenate/4303
  t34/80 -> concatenate/4304
  t34/81 -> concatenate/4305
  t34/82 -> concatenate/4306
  t34/83 -> concatenate/4307
  t34/84 -> concatenate/4308
  t34/85 -> concatenate/4309
  t34/86 -> concatenate/4310
  t34/87 -> concatenate/4311
  t34/88 -> concatenate/4312
  t34/89 -> concatenate/4313
  t34/90 -> concatenate/4314
  t34/91 -> concatenate/4315
  t34/92 -> concatenate/4316
  t34/93 -> concatenate/4317
  t34/94 -> concatenate/4318
  t34/95 -> concatenate/4319
  t34/96 -> concatenate/4320
  t34/97 -> concatenate/4321
  t34/98 -> concatenate/4322
  t34/99 -> concatenate/4323
  t34/100 -> concatenate/4324
  t34/101 -> concatenate/4325
  t34/102 -> concatenate/4326
  t34/103 -> concatenate/4327
  t34/104 -> concatenate/4328
  t34/105 -> concatenate/4329
  t34/106 -> concatenate/4330
  t34/107 -> concatenate/4331
  t34/108 -> concatenate/4332
  t34/109 -> concatenate/4333
  t34/110 -> concatenate/4334
  t34/111 -> concatenate/4335
  t34/112 -> concatenate/4336
  t34/113 -> concatenate/4337
  t34/114 -> concatenate/4338
  t34/115 -> concatenate/4339
  t34/116 -> concatenate/4340
  t34/117 -> concatenate/4341
  t34/118 -> concatenate/4342
  t34/119 -> concatenate/4343
  t34/120 -> concatenate/4344
  t34/121 -> concatenate/4345
  t34/122 -> concatenate/4346
  t34/123 -> concatenate/4347
  t34/124 -> concatenate/4348
  t34/125 -> concatenate/4349
  t34/126 -> concatenate/4350
  t34/127 -> concatenate/4351
  t34/128 -> concatenate/4352
  t35/1 -> concatenate/4353
  t35/2 -> concatenate/4354
  t35/3 -> concatenate/4355
  t35/4 -> concatenate/4356
  t35/5 -> concatenate/4357
  t35/6 -> concatenate/4358
  t35/7 -> concatenate/4359
  t35/8 -> concatenate/4360
  t35/9 -> concatenate/4361
  t35/10 -> concatenate/4362
  t35/11 -> concatenate/4363
  t35/12 -> concatenate/4364
  t35/13 -> concatenate/4365
  t35/14 -> concatenate/4366
  t35/15 -> concatenate/4367
  t35/16 -> concatenate/4368
  t35/17 -> concatenate/4369
  t35/18 -> concatenate/4370
  t35/19 -> concatenate/4371
  t35/20 -> concatenate/4372
  t35/21 -> concatenate/4373
  t35/22 -> concatenate/4374
  t35/23 -> concatenate/4375
  t35/24 -> concatenate/4376
  t35/25 -> concatenate/4377
  t35/26 -> concatenate/4378
  t35/27 -> concatenate/4379
  t35/28 -> concatenate/4380
  t35/29 -> concatenate/4381
  t35/30 -> concatenate/4382
  t35/31 -> concatenate/4383
  t35/32 -> concatenate/4384
  t35/33 -> concatenate/4385
  t35/34 -> concatenate/4386
  t35/35 -> concatenate/4387
  t35/36 -> concatenate/4388
  t35/37 -> concatenate/4389
  t35/38 -> concatenate/4390
  t35/39 -> concatenate/4391
  t35/40 -> concatenate/4392
  t35/41 -> concatenate/4393
  t35/42 -> concatenate/4394
  t35/43 -> concatenate/4395
  t35/44 -> concatenate/4396
  t35/45 -> concatenate/4397
  t35/46 -> concatenate/4398
  t35/47 -> concatenate/4399
  t35/48 -> concatenate/4400
  t35/49 -> concatenate/4401
  t35/50 -> concatenate/4402
  t35/51 -> concatenate/4403
  t35/52 -> concatenate/4404
  t35/53 -> concatenate/4405
  t35/54 -> concatenate/4406
  t35/55 -> concatenate/4407
  t35/56 -> concatenate/4408
  t35/57 -> concatenate/4409
  t35/58 -> concatenate/4410
  t35/59 -> concatenate/4411
  t35/60 -> concatenate/4412
  t35/61 -> concatenate/4413
  t35/62 -> concatenate/4414
  t35/63 -> concatenate/4415
  t35/64 -> concatenate/4416
  t35/65 -> concatenate/4417
  t35/66 -> concatenate/4418
  t35/67 -> concatenate/4419
  t35/68 -> concatenate/4420
  t35/69 -> concatenate/4421
  t35/70 -> concatenate/4422
  t35/71 -> concatenate/4423
  t35/72 -> concatenate/4424
  t35/73 -> concatenate/4425
  t35/74 -> concatenate/4426
  t35/75 -> concatenate/4427
  t35/76 -> concatenate/4428
  t35/77 -> concatenate/4429
  t35/78 -> concatenate/4430
  t35/79 -> concatenate/4431
  t35/80 -> concatenate/4432
  t35/81 -> concatenate/4433
  t35/82 -> concatenate/4434
  t35/83 -> concatenate/4435
  t35/84 -> concatenate/4436
  t35/85 -> concatenate/4437
  t35/86 -> concatenate/4438
  t35/87 -> concatenate/4439
  t35/88 -> concatenate/4440
  t35/89 -> concatenate/4441
  t35/90 -> concatenate/4442
  t35/91 -> concatenate/4443
  t35/92 -> concatenate/4444
  t35/93 -> concatenate/4445
  t35/94 -> concatenate/4446
  t35/95 -> concatenate/4447
  t35/96 -> concatenate/4448
  t35/97 -> concatenate/4449
  t35/98 -> concatenate/4450
  t35/99 -> concatenate/4451
  t35/100 -> concatenate/4452
  t35/101 -> concatenate/4453
  t35/102 -> concatenate/4454
  t35/103 -> concatenate/4455
  t35/104 -> concatenate/4456
  t35/105 -> concatenate/4457
  t35/106 -> concatenate/4458
  t35/107 -> concatenate/4459
  t35/108 -> concatenate/4460
  t35/109 -> concatenate/4461
  t35/110 -> concatenate/4462
  t35/111 -> concatenate/4463
  t35/112 -> concatenate/4464
  t35/113 -> concatenate/4465
  t35/114 -> concatenate/4466
  t35/115 -> concatenate/4467
  t35/116 -> concatenate/4468
  t35/117 -> concatenate/4469
  t35/118 -> concatenate/4470
  t35/119 -> concatenate/4471
  t35/120 -> concatenate/4472
  t35/121 -> concatenate/4473
  t35/122 -> concatenate/4474
  t35/123 -> concatenate/4475
  t35/124 -> concatenate/4476
  t35/125 -> concatenate/4477
  t35/126 -> concatenate/4478
  t35/127 -> concatenate/4479
  t35/128 -> concatenate/4480
  t36/1 -> concatenate/4481
  t36/2 -> concatenate/4482
  t36/3 -> concatenate/4483
  t36/4 -> concatenate/4484
  t36/5 -> concatenate/4485
  t36/6 -> concatenate/4486
  t36/7 -> concatenate/4487
  t36/8 -> concatenate/4488
  t36/9 -> concatenate/4489
  t36/10 -> concatenate/4490
  t36/11 -> concatenate/4491
  t36/12 -> concatenate/4492
  t36/13 -> concatenate/4493
  t36/14 -> concatenate/4494
  t36/15 -> concatenate/4495
  t36/16 -> concatenate/4496
  t36/17 -> concatenate/4497
  t36/18 -> concatenate/4498
  t36/19 -> concatenate/4499
  t36/20 -> concatenate/4500
  t36/21 -> concatenate/4501
  t36/22 -> concatenate/4502
  t36/23 -> concatenate/4503
  t36/24 -> concatenate/4504
  t36/25 -> concatenate/4505
  t36/26 -> concatenate/4506
  t36/27 -> concatenate/4507
  t36/28 -> concatenate/4508
  t36/29 -> concatenate/4509
  t36/30 -> concatenate/4510
  t36/31 -> concatenate/4511
  t36/32 -> concatenate/4512
  t36/33 -> concatenate/4513
  t36/34 -> concatenate/4514
  t36/35 -> concatenate/4515
  t36/36 -> concatenate/4516
  t36/37 -> concatenate/4517
  t36/38 -> concatenate/4518
  t36/39 -> concatenate/4519
  t36/40 -> concatenate/4520
  t36/41 -> concatenate/4521
  t36/42 -> concatenate/4522
  t36/43 -> concatenate/4523
  t36/44 -> concatenate/4524
  t36/45 -> concatenate/4525
  t36/46 -> concatenate/4526
  t36/47 -> concatenate/4527
  t36/48 -> concatenate/4528
  t36/49 -> concatenate/4529
  t36/50 -> concatenate/4530
  t36/51 -> concatenate/4531
  t36/52 -> concatenate/4532
  t36/53 -> concatenate/4533
  t36/54 -> concatenate/4534
  t36/55 -> concatenate/4535
  t36/56 -> concatenate/4536
  t36/57 -> concatenate/4537
  t36/58 -> concatenate/4538
  t36/59 -> concatenate/4539
  t36/60 -> concatenate/4540
  t36/61 -> concatenate/4541
  t36/62 -> concatenate/4542
  t36/63 -> concatenate/4543
  t36/64 -> concatenate/4544
  t36/65 -> concatenate/4545
  t36/66 -> concatenate/4546
  t36/67 -> concatenate/4547
  t36/68 -> concatenate/4548
  t36/69 -> concatenate/4549
  t36/70 -> concatenate/4550
  t36/71 -> concatenate/4551
  t36/72 -> concatenate/4552
  t36/73 -> concatenate/4553
  t36/74 -> concatenate/4554
  t36/75 -> concatenate/4555
  t36/76 -> concatenate/4556
  t36/77 -> concatenate/4557
  t36/78 -> concatenate/4558
  t36/79 -> concatenate/4559
  t36/80 -> concatenate/4560
  t36/81 -> concatenate/4561
  t36/82 -> concatenate/4562
  t36/83 -> concatenate/4563
  t36/84 -> concatenate/4564
  t36/85 -> concatenate/4565
  t36/86 -> concatenate/4566
  t36/87 -> concatenate/4567
  t36/88 -> concatenate/4568
  t36/89 -> concatenate/4569
  t36/90 -> concatenate/4570
  t36/91 -> concatenate/4571
  t36/92 -> concatenate/4572
  t36/93 -> concatenate/4573
  t36/94 -> concatenate/4574
  t36/95 -> concatenate/4575
  t36/96 -> concatenate/4576
  t36/97 -> concatenate/4577
  t36/98 -> concatenate/4578
  t36/99 -> concatenate/4579
  t36/100 -> concatenate/4580
  t36/101 -> concatenate/4581
  t36/102 -> concatenate/4582
  t36/103 -> concatenate/4583
  t36/104 -> concatenate/4584
  t36/105 -> concatenate/4585
  t36/106 -> concatenate/4586
  t36/107 -> concatenate/4587
  t36/108 -> concatenate/4588
  t36/109 -> concatenate/4589
  t36/110 -> concatenate/4590
  t36/111 -> concatenate/4591
  t36/112 -> concatenate/4592
  t36/113 -> concatenate/4593
  t36/114 -> concatenate/4594
  t36/115 -> concatenate/4595
  t36/116 -> concatenate/4596
  t36/117 -> concatenate/4597
  t36/118 -> concatenate/4598
  t36/119 -> concatenate/4599
  t36/120 -> concatenate/4600
  t36/121 -> concatenate/4601
  t36/122 -> concatenate/4602
  t36/123 -> concatenate/4603
  t36/124 -> concatenate/4604
  t36/125 -> concatenate/4605
  t36/126 -> concatenate/4606
  t36/127 -> concatenate/4607
  t36/128 -> concatenate/4608
  t37/1 -> concatenate/4609
  t37/2 -> concatenate/4610
  t37/3 -> concatenate/4611
  t37/4 -> concatenate/4612
  t37/5 -> concatenate/4613
  t37/6 -> concatenate/4614
  t37/7 -> concatenate/4615
  t37/8 -> concatenate/4616
  t37/9 -> concatenate/4617
  t37/10 -> concatenate/4618
  t37/11 -> concatenate/4619
  t37/12 -> concatenate/4620
  t37/13 -> concatenate/4621
  t37/14 -> concatenate/4622
  t37/15 -> concatenate/4623
  t37/16 -> concatenate/4624
  t37/17 -> concatenate/4625
  t37/18 -> concatenate/4626
  t37/19 -> concatenate/4627
  t37/20 -> concatenate/4628
  t37/21 -> concatenate/4629
  t37/22 -> concatenate/4630
  t37/23 -> concatenate/4631
  t37/24 -> concatenate/4632
  t37/25 -> concatenate/4633
  t37/26 -> concatenate/4634
  t37/27 -> concatenate/4635
  t37/28 -> concatenate/4636
  t37/29 -> concatenate/4637
  t37/30 -> concatenate/4638
  t37/31 -> concatenate/4639
  t37/32 -> concatenate/4640
  t37/33 -> concatenate/4641
  t37/34 -> concatenate/4642
  t37/35 -> concatenate/4643
  t37/36 -> concatenate/4644
  t37/37 -> concatenate/4645
  t37/38 -> concatenate/4646
  t37/39 -> concatenate/4647
  t37/40 -> concatenate/4648
  t37/41 -> concatenate/4649
  t37/42 -> concatenate/4650
  t37/43 -> concatenate/4651
  t37/44 -> concatenate/4652
  t37/45 -> concatenate/4653
  t37/46 -> concatenate/4654
  t37/47 -> concatenate/4655
  t37/48 -> concatenate/4656
  t37/49 -> concatenate/4657
  t37/50 -> concatenate/4658
  t37/51 -> concatenate/4659
  t37/52 -> concatenate/4660
  t37/53 -> concatenate/4661
  t37/54 -> concatenate/4662
  t37/55 -> concatenate/4663
  t37/56 -> concatenate/4664
  t37/57 -> concatenate/4665
  t37/58 -> concatenate/4666
  t37/59 -> concatenate/4667
  t37/60 -> concatenate/4668
  t37/61 -> concatenate/4669
  t37/62 -> concatenate/4670
  t37/63 -> concatenate/4671
  t37/64 -> concatenate/4672
  t37/65 -> concatenate/4673
  t37/66 -> concatenate/4674
  t37/67 -> concatenate/4675
  t37/68 -> concatenate/4676
  t37/69 -> concatenate/4677
  t37/70 -> concatenate/4678
  t37/71 -> concatenate/4679
  t37/72 -> concatenate/4680
  t37/73 -> concatenate/4681
  t37/74 -> concatenate/4682
  t37/75 -> concatenate/4683
  t37/76 -> concatenate/4684
  t37/77 -> concatenate/4685
  t37/78 -> concatenate/4686
  t37/79 -> concatenate/4687
  t37/80 -> concatenate/4688
  t37/81 -> concatenate/4689
  t37/82 -> concatenate/4690
  t37/83 -> concatenate/4691
  t37/84 -> concatenate/4692
  t37/85 -> concatenate/4693
  t37/86 -> concatenate/4694
  t37/87 -> concatenate/4695
  t37/88 -> concatenate/4696
  t37/89 -> concatenate/4697
  t37/90 -> concatenate/4698
  t37/91 -> concatenate/4699
  t37/92 -> concatenate/4700
  t37/93 -> concatenate/4701
  t37/94 -> concatenate/4702
  t37/95 -> concatenate/4703
  t37/96 -> concatenate/4704
  t37/97 -> concatenate/4705
  t37/98 -> concatenate/4706
  t37/99 -> concatenate/4707
  t37/100 -> concatenate/4708
  t37/101 -> concatenate/4709
  t37/102 -> concatenate/4710
  t37/103 -> concatenate/4711
  t37/104 -> concatenate/4712
  t37/105 -> concatenate/4713
  t37/106 -> concatenate/4714
  t37/107 -> concatenate/4715
  t37/108 -> concatenate/4716
  t37/109 -> concatenate/4717
  t37/110 -> concatenate/4718
  t37/111 -> concatenate/4719
  t37/112 -> concatenate/4720
  t37/113 -> concatenate/4721
  t37/114 -> concatenate/4722
  t37/115 -> concatenate/4723
  t37/116 -> concatenate/4724
  t37/117 -> concatenate/4725
  t37/118 -> concatenate/4726
  t37/119 -> concatenate/4727
  t37/120 -> concatenate/4728
  t37/121 -> concatenate/4729
  t37/122 -> concatenate/4730
  t37/123 -> concatenate/4731
  t37/124 -> concatenate/4732
  t37/125 -> concatenate/4733
  t37/126 -> concatenate/4734
  t37/127 -> concatenate/4735
  t37/128 -> concatenate/4736
  t38/1 -> concatenate/4737
  t38/2 -> concatenate/4738
  t38/3 -> concatenate/4739
  t38/4 -> concatenate/4740
  t38/5 -> concatenate/4741
  t38/6 -> concatenate/4742
  t38/7 -> concatenate/4743
  t38/8 -> concatenate/4744
  t38/9 -> concatenate/4745
  t38/10 -> concatenate/4746
  t38/11 -> concatenate/4747
  t38/12 -> concatenate/4748
  t38/13 -> concatenate/4749
  t38/14 -> concatenate/4750
  t38/15 -> concatenate/4751
  t38/16 -> concatenate/4752
  t38/17 -> concatenate/4753
  t38/18 -> concatenate/4754
  t38/19 -> concatenate/4755
  t38/20 -> concatenate/4756
  t38/21 -> concatenate/4757
  t38/22 -> concatenate/4758
  t38/23 -> concatenate/4759
  t38/24 -> concatenate/4760
  t38/25 -> concatenate/4761
  t38/26 -> concatenate/4762
  t38/27 -> concatenate/4763
  t38/28 -> concatenate/4764
  t38/29 -> concatenate/4765
  t38/30 -> concatenate/4766
  t38/31 -> concatenate/4767
  t38/32 -> concatenate/4768
  t38/33 -> concatenate/4769
  t38/34 -> concatenate/4770
  t38/35 -> concatenate/4771
  t38/36 -> concatenate/4772
  t38/37 -> concatenate/4773
  t38/38 -> concatenate/4774
  t38/39 -> concatenate/4775
  t38/40 -> concatenate/4776
  t38/41 -> concatenate/4777
  t38/42 -> concatenate/4778
  t38/43 -> concatenate/4779
  t38/44 -> concatenate/4780
  t38/45 -> concatenate/4781
  t38/46 -> concatenate/4782
  t38/47 -> concatenate/4783
  t38/48 -> concatenate/4784
  t38/49 -> concatenate/4785
  t38/50 -> concatenate/4786
  t38/51 -> concatenate/4787
  t38/52 -> concatenate/4788
